simulink model "frb_stable_test"  (R2013b)
(part 3 of 48)

      mask help: This simple vector accumulator is based on a shift register. It outputs its previous accumulated vector after a new_acc pulse is received.
      mask init:
      | simple_bram_vacc_init(gcb, ...
      |     'vec_len', vec_len, ...
      |     'arith_type', arith_type, ...
      |     'n_bits', n_bits, ...
      |     'bin_pt', bin_pt);
      mask TypeOptions arith_type: Signed | Unsigned
  simple_bram_vacc45 : Subsystem  AncestorBlock=casper_library_accumulators/simple_bram_vacc  mask(simple_bram_vacc){vec_len=512, arith_type=Unsigned, n_bits=32, bin_pt=19}
      mask prompts: vec_len "Vector length:"; arith_type "Output type:"; n_bits "Bit width (output):"; bin_pt "Binary point (output):"
      mask help: This simple vector accumulator is based on a shift register. It outputs its previous accumulated vector after a new_acc pulse is received.
      mask init:
      | simple_bram_vacc_init(gcb, ...
      |     'vec_len', vec_len, ...
      |     'arith_type', arith_type, ...
      |     'n_bits', n_bits, ...
      |     'bin_pt', bin_pt);
      mask TypeOptions arith_type: Signed | Unsigned
  simple_bram_vacc46 : Subsystem  AncestorBlock=casper_library_accumulators/simple_bram_vacc  mask(simple_bram_vacc){vec_len=512, arith_type=Unsigned, n_bits=32, bin_pt=19}
      mask prompts: vec_len "Vector length:"; arith_type "Output type:"; n_bits "Bit width (output):"; bin_pt "Binary point (output):"
      mask help: This simple vector accumulator is based on a shift register. It outputs its previous accumulated vector after a new_acc pulse is received.
      mask init:
      | simple_bram_vacc_init(gcb, ...
      |     'vec_len', vec_len, ...
      |     'arith_type', arith_type, ...
      |     'n_bits', n_bits, ...
      |     'bin_pt', bin_pt);
      mask TypeOptions arith_type: Signed | Unsigned
  simple_bram_vacc5 : Subsystem  AncestorBlock=casper_library_accumulators/simple_bram_vacc  mask(simple_bram_vacc){vec_len=512, arith_type=Unsigned, n_bits=32, bin_pt=19}
      mask prompts: vec_len "Vector length:"; arith_type "Output type:"; n_bits "Bit width (output):"; bin_pt "Binary point (output):"
      mask help: This simple vector accumulator is based on a shift register. It outputs its previous accumulated vector after a new_acc pulse is received.
      mask init:
      | simple_bram_vacc_init(gcb, ...
      |     'vec_len', vec_len, ...
      |     'arith_type', arith_type, ...
      |     'n_bits', n_bits, ...
      |     'bin_pt', bin_pt);
      mask TypeOptions arith_type: Signed | Unsigned
  simple_bram_vacc6 : Subsystem  AncestorBlock=casper_library_accumulators/simple_bram_vacc  mask(simple_bram_vacc){vec_len=512, arith_type=Unsigned, n_bits=32, bin_pt=19}
      mask prompts: vec_len "Vector length:"; arith_type "Output type:"; n_bits "Bit width (output):"; bin_pt "Binary point (output):"
      mask help: This simple vector accumulator is based on a shift register. It outputs its previous accumulated vector after a new_acc pulse is received.
      mask init:
      | simple_bram_vacc_init(gcb, ...
      |     'vec_len', vec_len, ...
      |     'arith_type', arith_type, ...
      |     'n_bits', n_bits, ...
      |     'bin_pt', bin_pt);
      mask TypeOptions arith_type: Signed | Unsigned
  simple_bram_vacc7 : Subsystem  AncestorBlock=casper_library_accumulators/simple_bram_vacc  mask(simple_bram_vacc){vec_len=512, arith_type=Unsigned, n_bits=32, bin_pt=19}
      mask prompts: vec_len "Vector length:"; arith_type "Output type:"; n_bits "Bit width (output):"; bin_pt "Binary point (output):"
      mask help: This simple vector accumulator is based on a shift register. It outputs its previous accumulated vector after a new_acc pulse is received.
      mask init:
      | simple_bram_vacc_init(gcb, ...
      |     'vec_len', vec_len, ...
      |     'arith_type', arith_type, ...
      |     'n_bits', n_bits, ...
      |     'bin_pt', bin_pt);
      mask TypeOptions arith_type: Signed | Unsigned
  simple_bram_vacc8 : Subsystem  AncestorBlock=casper_library_accumulators/simple_bram_vacc  mask(simple_bram_vacc){vec_len=512, arith_type=Unsigned, n_bits=32, bin_pt=19}
      mask prompts: vec_len "Vector length:"; arith_type "Output type:"; n_bits "Bit width (output):"; bin_pt "Binary point (output):"
      mask help: This simple vector accumulator is based on a shift register. It outputs its previous accumulated vector after a new_acc pulse is received.
      mask init:
      | simple_bram_vacc_init(gcb, ...
      |     'vec_len', vec_len, ...
      |     'arith_type', arith_type, ...
      |     'n_bits', n_bits, ...
      |     'bin_pt', bin_pt);
      mask TypeOptions arith_type: Signed | Unsigned
  simple_bram_vacc9 : Subsystem  AncestorBlock=casper_library_accumulators/simple_bram_vacc  mask(simple_bram_vacc){vec_len=512, arith_type=Unsigned, n_bits=32, bin_pt=19}
      mask prompts: vec_len "Vector length:"; arith_type "Output type:"; n_bits "Bit width (output):"; bin_pt "Binary point (output):"
      mask help: This simple vector accumulator is based on a shift register. It outputs its previous accumulated vector after a new_acc pulse is received.
      mask init:
      | simple_bram_vacc_init(gcb, ...
      |     'vec_len', vec_len, ...
      |     'arith_type', arith_type, ...
      |     'n_bits', n_bits, ...
      |     'bin_pt', bin_pt);
      mask TypeOptions arith_type: Signed | Unsigned
  simple_bram_vacc_0a_1 : Subsystem  AncestorBlock=casper_library_accumulators/simple_bram_vacc  mask(simple_bram_vacc){vec_len=512, arith_type=Unsigned, n_bits=32, bin_pt=16}
      mask prompts: vec_len "Vector length:"; arith_type "Output type:"; n_bits "Bit width (output):"; bin_pt "Binary point (output):"
      mask help: This simple vector accumulator is based on a shift register. It outputs its previous accumulated vector after a new_acc pulse is received.
      mask init:
      | simple_bram_vacc_init(gcb, ...
      |     'vec_len', vec_len, ...
      |     'arith_type', arith_type, ...
      |     'n_bits', n_bits, ...
      |     'bin_pt', bin_pt);
      mask TypeOptions arith_type: Signed | Unsigned
  simple_bram_vacc_0a_2 : Subsystem  AncestorBlock=casper_library_accumulators/simple_bram_vacc  mask(simple_bram_vacc){vec_len=512, arith_type=Unsigned, n_bits=32, bin_pt=16}
      mask prompts: vec_len "Vector length:"; arith_type "Output type:"; n_bits "Bit width (output):"; bin_pt "Binary point (output):"
      mask help: This simple vector accumulator is based on a shift register. It outputs its previous accumulated vector after a new_acc pulse is received.
      mask init:
      | simple_bram_vacc_init(gcb, ...
      |     'vec_len', vec_len, ...
      |     'arith_type', arith_type, ...
      |     'n_bits', n_bits, ...
      |     'bin_pt', bin_pt);
      mask TypeOptions arith_type: Signed | Unsigned
  simple_bram_vacc_0a_3 : Subsystem  AncestorBlock=casper_library_accumulators/simple_bram_vacc  mask(simple_bram_vacc){vec_len=512, arith_type=Unsigned, n_bits=32, bin_pt=16}
      mask prompts: vec_len "Vector length:"; arith_type "Output type:"; n_bits "Bit width (output):"; bin_pt "Binary point (output):"
      mask help: This simple vector accumulator is based on a shift register. It outputs its previous accumulated vector after a new_acc pulse is received.
      mask init:
      | simple_bram_vacc_init(gcb, ...
      |     'vec_len', vec_len, ...
      |     'arith_type', arith_type, ...
      |     'n_bits', n_bits, ...
      |     'bin_pt', bin_pt);
      mask TypeOptions arith_type: Signed | Unsigned
  simple_bram_vacc_0a_8 : Subsystem  AncestorBlock=casper_library_accumulators/simple_bram_vacc  mask(simple_bram_vacc){vec_len=512, arith_type=Unsigned, n_bits=32, bin_pt=16}
      mask prompts: vec_len "Vector length:"; arith_type "Output type:"; n_bits "Bit width (output):"; bin_pt "Binary point (output):"
      mask help: This simple vector accumulator is based on a shift register. It outputs its previous accumulated vector after a new_acc pulse is received.
      mask init:
      | simple_bram_vacc_init(gcb, ...
      |     'vec_len', vec_len, ...
      |     'arith_type', arith_type, ...
      |     'n_bits', n_bits, ...
      |     'bin_pt', bin_pt);
      mask TypeOptions arith_type: Signed | Unsigned
  simple_bram_vacc_0c_16 : Subsystem  AncestorBlock=casper_library_accumulators/simple_bram_vacc  mask(simple_bram_vacc){vec_len=512, arith_type=Signed, n_bits=32, bin_pt=16}
      mask prompts: vec_len "Vector length:"; arith_type "Output type:"; n_bits "Bit width (output):"; bin_pt "Binary point (output):"
      mask help: This simple vector accumulator is based on a shift register. It outputs its previous accumulated vector after a new_acc pulse is received.
      mask init:
      | simple_bram_vacc_init(gcb, ...
      |     'vec_len', vec_len, ...
      |     'arith_type', arith_type, ...
      |     'n_bits', n_bits, ...
      |     'bin_pt', bin_pt);
      mask TypeOptions arith_type: Signed | Unsigned
  simple_bram_vacc_0c_17 : Subsystem  AncestorBlock=casper_library_accumulators/simple_bram_vacc  mask(simple_bram_vacc){vec_len=512, arith_type=Signed, n_bits=32, bin_pt=16}
      mask prompts: vec_len "Vector length:"; arith_type "Output type:"; n_bits "Bit width (output):"; bin_pt "Binary point (output):"
      mask help: This simple vector accumulator is based on a shift register. It outputs its previous accumulated vector after a new_acc pulse is received.
      mask init:
      | simple_bram_vacc_init(gcb, ...
      |     'vec_len', vec_len, ...
      |     'arith_type', arith_type, ...
      |     'n_bits', n_bits, ...
      |     'bin_pt', bin_pt);
      mask TypeOptions arith_type: Signed | Unsigned
  simple_bram_vacc_0c_18 : Subsystem  AncestorBlock=casper_library_accumulators/simple_bram_vacc  mask(simple_bram_vacc){vec_len=512, arith_type=Signed, n_bits=32, bin_pt=16}
      mask prompts: vec_len "Vector length:"; arith_type "Output type:"; n_bits "Bit width (output):"; bin_pt "Binary point (output):"
      mask help: This simple vector accumulator is based on a shift register. It outputs its previous accumulated vector after a new_acc pulse is received.
      mask init:
      | simple_bram_vacc_init(gcb, ...
      |     'vec_len', vec_len, ...
      |     'arith_type', arith_type, ...
      |     'n_bits', n_bits, ...
      |     'bin_pt', bin_pt);
      mask TypeOptions arith_type: Signed | Unsigned
  simple_bram_vacc_0c_19 : Subsystem  AncestorBlock=casper_library_accumulators/simple_bram_vacc  mask(simple_bram_vacc){vec_len=512, arith_type=Signed, n_bits=32, bin_pt=16}
      mask prompts: vec_len "Vector length:"; arith_type "Output type:"; n_bits "Bit width (output):"; bin_pt "Binary point (output):"
      mask help: This simple vector accumulator is based on a shift register. It outputs its previous accumulated vector after a new_acc pulse is received.
      mask init:
      | simple_bram_vacc_init(gcb, ...
      |     'vec_len', vec_len, ...
      |     'arith_type', arith_type, ...
      |     'n_bits', n_bits, ...
      |     'bin_pt', bin_pt);
      mask TypeOptions arith_type: Signed | Unsigned
  simple_bram_vacc_0c_20 : Subsystem  AncestorBlock=casper_library_accumulators/simple_bram_vacc  mask(simple_bram_vacc){vec_len=512, arith_type=Unsigned, n_bits=32, bin_pt=16}
      mask prompts: vec_len "Vector length:"; arith_type "Output type:"; n_bits "Bit width (output):"; bin_pt "Binary point (output):"
      mask help: This simple vector accumulator is based on a shift register. It outputs its previous accumulated vector after a new_acc pulse is received.
      mask init:
      | simple_bram_vacc_init(gcb, ...
      |     'vec_len', vec_len, ...
      |     'arith_type', arith_type, ...
      |     'n_bits', n_bits, ...
      |     'bin_pt', bin_pt);
      mask TypeOptions arith_type: Signed | Unsigned
  simple_bram_vacc_0c_21 : Subsystem  AncestorBlock=casper_library_accumulators/simple_bram_vacc  mask(simple_bram_vacc){vec_len=512, arith_type=Unsigned, n_bits=32, bin_pt=16}
      mask prompts: vec_len "Vector length:"; arith_type "Output type:"; n_bits "Bit width (output):"; bin_pt "Binary point (output):"
      mask help: This simple vector accumulator is based on a shift register. It outputs its previous accumulated vector after a new_acc pulse is received.
      mask init:
      | simple_bram_vacc_init(gcb, ...
      |     'vec_len', vec_len, ...
      |     'arith_type', arith_type, ...
      |     'n_bits', n_bits, ...
      |     'bin_pt', bin_pt);
      mask TypeOptions arith_type: Signed | Unsigned
  simple_bram_vacc_0c_22 : Subsystem  AncestorBlock=casper_library_accumulators/simple_bram_vacc  mask(simple_bram_vacc){vec_len=512, arith_type=Signed, n_bits=32, bin_pt=16}
      mask prompts: vec_len "Vector length:"; arith_type "Output type:"; n_bits "Bit width (output):"; bin_pt "Binary point (output):"
      mask help: This simple vector accumulator is based on a shift register. It outputs its previous accumulated vector after a new_acc pulse is received.
      mask init:
      | simple_bram_vacc_init(gcb, ...
      |     'vec_len', vec_len, ...
      |     'arith_type', arith_type, ...
      |     'n_bits', n_bits, ...
      |     'bin_pt', bin_pt);
      mask TypeOptions arith_type: Signed | Unsigned
  simple_bram_vacc_0c_23 : Subsystem  AncestorBlock=casper_library_accumulators/simple_bram_vacc  mask(simple_bram_vacc){vec_len=512, arith_type=Signed, n_bits=32, bin_pt=16}
      mask prompts: vec_len "Vector length:"; arith_type "Output type:"; n_bits "Bit width (output):"; bin_pt "Binary point (output):"
      mask help: This simple vector accumulator is based on a shift register. It outputs its previous accumulated vector after a new_acc pulse is received.
      mask init:
      | simple_bram_vacc_init(gcb, ...
      |     'vec_len', vec_len, ...
      |     'arith_type', arith_type, ...
      |     'n_bits', n_bits, ...
      |     'bin_pt', bin_pt);
      mask TypeOptions arith_type: Signed | Unsigned
  simple_bram_vacc_0c_4 : Subsystem  AncestorBlock=casper_library_accumulators/simple_bram_vacc  mask(simple_bram_vacc){vec_len=512, arith_type=Unsigned, n_bits=32, bin_pt=16}
      mask prompts: vec_len "Vector length:"; arith_type "Output type:"; n_bits "Bit width (output):"; bin_pt "Binary point (output):"
      mask help: This simple vector accumulator is based on a shift register. It outputs its previous accumulated vector after a new_acc pulse is received.
      mask init:
      | simple_bram_vacc_init(gcb, ...
      |     'vec_len', vec_len, ...
      |     'arith_type', arith_type, ...
      |     'n_bits', n_bits, ...
      |     'bin_pt', bin_pt);
      mask TypeOptions arith_type: Signed | Unsigned
  simple_bram_vacc_0c_5 : Subsystem  AncestorBlock=casper_library_accumulators/simple_bram_vacc  mask(simple_bram_vacc){vec_len=512, arith_type=Unsigned, n_bits=32, bin_pt=16}
      mask prompts: vec_len "Vector length:"; arith_type "Output type:"; n_bits "Bit width (output):"; bin_pt "Binary point (output):"
      mask help: This simple vector accumulator is based on a shift register. It outputs its previous accumulated vector after a new_acc pulse is received.
      mask init:
      | simple_bram_vacc_init(gcb, ...
      |     'vec_len', vec_len, ...
      |     'arith_type', arith_type, ...
      |     'n_bits', n_bits, ...
      |     'bin_pt', bin_pt);
      mask TypeOptions arith_type: Signed | Unsigned
  simple_bram_vacc_0c_6 : Subsystem  AncestorBlock=casper_library_accumulators/simple_bram_vacc  mask(simple_bram_vacc){vec_len=512, arith_type=Signed, n_bits=32, bin_pt=16}
      mask prompts: vec_len "Vector length:"; arith_type "Output type:"; n_bits "Bit width (output):"; bin_pt "Binary point (output):"
      mask help: This simple vector accumulator is based on a shift register. It outputs its previous accumulated vector after a new_acc pulse is received.
      mask init:
      | simple_bram_vacc_init(gcb, ...
      |     'vec_len', vec_len, ...
      |     'arith_type', arith_type, ...
      |     'n_bits', n_bits, ...
      |     'bin_pt', bin_pt);
      mask TypeOptions arith_type: Signed | Unsigned
  simple_bram_vacc_0c_7 : Subsystem  AncestorBlock=casper_library_accumulators/simple_bram_vacc  mask(simple_bram_vacc){vec_len=512, arith_type=Signed, n_bits=32, bin_pt=16}
      mask prompts: vec_len "Vector length:"; arith_type "Output type:"; n_bits "Bit width (output):"; bin_pt "Binary point (output):"
      mask help: This simple vector accumulator is based on a shift register. It outputs its previous accumulated vector after a new_acc pulse is received.
      mask init:
      | simple_bram_vacc_init(gcb, ...
      |     'vec_len', vec_len, ...
      |     'arith_type', arith_type, ...
      |     'n_bits', n_bits, ...
      |     'bin_pt', bin_pt);
      mask TypeOptions arith_type: Signed | Unsigned
  small_spec2 : Subsystem  Tag=xps:bram  AncestorBlock=xps_library/Shared_BRAM  mask{arith_type=Unsigned, addr_width=10, data_width=32, reg_prim_output=off, reg_core_output=off, optimization=Minimum_Area, data_bin_pt=0, init_vals=[0:2^10-1], sample_rate=1}
      mask prompts: arith_type "Output Data Type"; addr_width "Address width"; data_width "Data Width"; reg_prim_output "Register Primitive Output"; reg_core_output "Register Core Output"; data_bin_pt "Data Binary Point"; init_vals "Initial values (simulation only)"; sample_rate "Sample rate"
      mask init:
      | shared_bram_mask;
      mask TypeOptions arith_type: Unsigned | Signed  (2's comp)
      mask TypeOptions data_width: 8 | 16 | 32 | 64 | 128
      mask TypeOptions optimization: Minimum_Area | Low_Power
  snapshot : Subsystem  Tag=casper:snapshot  AncestorBlock=casper_library_scopes/snapshot  mask(snapshot){storage=bram, dram_dimm=1, dram_clock=200, nsamples=10, data_width=64, offset=off, circap=off, value=off, use_dsp48=off}
      mask prompts: storage "Storage medium"; dram_dimm "DRAM dimm"; dram_clock "DRAM clock rate"; nsamples "Number of Samples (2^?)"; data_width "Data width"; offset "Start delay support"; circap "Circular capture support"; value "Extra value capture support"; use_dsp48 "Use DSP48s to implement counters"
      mask help:
      | Standard snap block, but with the following optional extras;
      |  1) Optionally delay the fabric trigger by a user-specified number of valids.
      |  2) Capture continuously after a trigger until a stop pulse is received. Data is captured into BRAM continuously, with old data being overwritten until a stop command is received. Then stop capturing when memory is filled. This enables you to get some data before and some data after the stop pulse. Use the 'tr_en_cnt' register to determine where you are in your vector. 'Addr' register's MSb now indicates 'busy capturing'.
      |  3) Optionally capture a value on an input port to a register at the same time as the first data sample.
      |  4) Implement counters using DSP48Es to save resources.
      mask init: same as frb_stable_test/adcsnap1
      mask TypeOptions storage: bram | dram
      mask Callback storage: snapshot_callback();
      mask TypeOptions dram_dimm: 1 | 2 | 3 | 4
      mask TypeOptions dram_clock: 200 | 250 | 266 | 300 | 333
      mask TypeOptions data_width: 8 | 16 | 32 | 64 | 128
  spec1_0 : Subsystem  Tag=xps:bram  AncestorBlock=xps_library/Shared_BRAM  mask{arith_type=Unsigned, addr_width=9, data_width=64, reg_prim_output=on, reg_core_output=on, optimization=Minimum_Area, data_bin_pt=0, init_vals=[0:2^10-1], sample_rate=1}
      mask prompts: arith_type "Output Data Type"; addr_width "Address width"; data_width "Data Width"; reg_prim_output "Register Primitive Output"; reg_core_output "Register Core Output"; data_bin_pt "Data Binary Point"; init_vals "Initial values (simulation only)"; sample_rate "Sample rate"
      mask init:
      | shared_bram_mask;
      mask TypeOptions arith_type: Unsigned | Signed  (2's comp)
      mask TypeOptions data_width: 8 | 16 | 32 | 64 | 128
      mask TypeOptions optimization: Minimum_Area | Low_Power
  spec1_1 : Subsystem  Tag=xps:bram  AncestorBlock=xps_library/Shared_BRAM  mask{arith_type=Unsigned, addr_width=9, data_width=64, reg_prim_output=on, reg_core_output=on, optimization=Minimum_Area, data_bin_pt=0, init_vals=[0:2^10-1], sample_rate=1}
      mask prompts: arith_type "Output Data Type"; addr_width "Address width"; data_width "Data Width"; reg_prim_output "Register Primitive Output"; reg_core_output "Register Core Output"; data_bin_pt "Data Binary Point"; init_vals "Initial values (simulation only)"; sample_rate "Sample rate"
      mask init:
      | shared_bram_mask;
      mask TypeOptions arith_type: Unsigned | Signed  (2's comp)
      mask TypeOptions data_width: 8 | 16 | 32 | 64 | 128
      mask TypeOptions optimization: Minimum_Area | Low_Power
  spec2_0 : Subsystem  Tag=xps:bram  AncestorBlock=xps_library/Shared_BRAM  mask{arith_type=Unsigned, addr_width=9, data_width=64, reg_prim_output=on, reg_core_output=on, optimization=Minimum_Area, data_bin_pt=0, init_vals=[0:2^10-1], sample_rate=1}
      mask prompts: arith_type "Output Data Type"; addr_width "Address width"; data_width "Data Width"; reg_prim_output "Register Primitive Output"; reg_core_output "Register Core Output"; data_bin_pt "Data Binary Point"; init_vals "Initial values (simulation only)"; sample_rate "Sample rate"
      mask init:
      | shared_bram_mask;
      mask TypeOptions arith_type: Unsigned | Signed  (2's comp)
      mask TypeOptions data_width: 8 | 16 | 32 | 64 | 128
      mask TypeOptions optimization: Minimum_Area | Low_Power
  spec2_1 : Subsystem  Tag=xps:bram  AncestorBlock=xps_library/Shared_BRAM  mask{arith_type=Unsigned, addr_width=9, data_width=64, reg_prim_output=on, reg_core_output=on, optimization=Minimum_Area, data_bin_pt=0, init_vals=[0:2^10-1], sample_rate=1}
      mask prompts: arith_type "Output Data Type"; addr_width "Address width"; data_width "Data Width"; reg_prim_output "Register Primitive Output"; reg_core_output "Register Core Output"; data_bin_pt "Data Binary Point"; init_vals "Initial values (simulation only)"; sample_rate "Sample rate"
      mask init:
      | shared_bram_mask;
      mask TypeOptions arith_type: Unsigned | Signed  (2's comp)
      mask TypeOptions data_width: 8 | 16 | 32 | 64 | 128
      mask TypeOptions optimization: Minimum_Area | Low_Power
  spec3_0 : Subsystem  Tag=xps:bram  AncestorBlock=xps_library/Shared_BRAM  mask{arith_type=Unsigned, addr_width=9, data_width=64, reg_prim_output=on, reg_core_output=on, optimization=Minimum_Area, data_bin_pt=0, init_vals=[0:2^10-1], sample_rate=1}
      mask prompts: arith_type "Output Data Type"; addr_width "Address width"; data_width "Data Width"; reg_prim_output "Register Primitive Output"; reg_core_output "Register Core Output"; data_bin_pt "Data Binary Point"; init_vals "Initial values (simulation only)"; sample_rate "Sample rate"
      mask init:
      | shared_bram_mask;
      mask TypeOptions arith_type: Unsigned | Signed  (2's comp)
      mask TypeOptions data_width: 8 | 16 | 32 | 64 | 128
      mask TypeOptions optimization: Minimum_Area | Low_Power
  spec3_1 : Subsystem  Tag=xps:bram  AncestorBlock=xps_library/Shared_BRAM  mask{arith_type=Unsigned, addr_width=9, data_width=64, reg_prim_output=on, reg_core_output=on, optimization=Minimum_Area, data_bin_pt=0, init_vals=[0:2^10-1], sample_rate=1}
      mask prompts: arith_type "Output Data Type"; addr_width "Address width"; data_width "Data Width"; reg_prim_output "Register Primitive Output"; reg_core_output "Register Core Output"; data_bin_pt "Data Binary Point"; init_vals "Initial values (simulation only)"; sample_rate "Sample rate"
      mask init:
      | shared_bram_mask;
      mask TypeOptions arith_type: Unsigned | Signed  (2's comp)
      mask TypeOptions data_width: 8 | 16 | 32 | 64 | 128
      mask TypeOptions optimization: Minimum_Area | Low_Power
  spec4_0 : Subsystem  Tag=xps:bram  AncestorBlock=xps_library/Shared_BRAM  mask{arith_type=Unsigned, addr_width=9, data_width=64, reg_prim_output=on, reg_core_output=on, optimization=Minimum_Area, data_bin_pt=0, init_vals=[0:2^10-1], sample_rate=1}
      mask prompts: arith_type "Output Data Type"; addr_width "Address width"; data_width "Data Width"; reg_prim_output "Register Primitive Output"; reg_core_output "Register Core Output"; data_bin_pt "Data Binary Point"; init_vals "Initial values (simulation only)"; sample_rate "Sample rate"
      mask init:
      | shared_bram_mask;
      mask TypeOptions arith_type: Unsigned | Signed  (2's comp)
      mask TypeOptions data_width: 8 | 16 | 32 | 64 | 128
      mask TypeOptions optimization: Minimum_Area | Low_Power
  spec4_1 : Subsystem  Tag=xps:bram  AncestorBlock=xps_library/Shared_BRAM  mask{arith_type=Unsigned, addr_width=9, data_width=64, reg_prim_output=on, reg_core_output=on, optimization=Minimum_Area, data_bin_pt=0, init_vals=[0:2^10-1], sample_rate=1}
      mask prompts: arith_type "Output Data Type"; addr_width "Address width"; data_width "Data Width"; reg_prim_output "Register Primitive Output"; reg_core_output "Register Core Output"; data_bin_pt "Data Binary Point"; init_vals "Initial values (simulation only)"; sample_rate "Sample rate"
      mask init:
      | shared_bram_mask;
      mask TypeOptions arith_type: Unsigned | Signed  (2's comp)
      mask TypeOptions data_width: 8 | 16 | 32 | 64 | 128
      mask TypeOptions optimization: Minimum_Area | Low_Power
  sync_gen : Subsystem  AncestorBlock=casper_library_misc/sync_gen  mask(sync_gen){sim_acc_len=1, fft_size=4096, fft_simult_inputs=8, pfb_fir_taps=3, reorder_vec=[2 2 9], scale=1}
      mask prompts: sim_acc_len "Simulation Accumulation Length"; fft_size "FFT Size"; fft_simult_inputs "Simultaneous Inputs (FFT)"; pfb_fir_taps "Taps in pfb_fir (use 1 if no pfb_fir)"; reorder_vec "Reorder Orders (e.g. [2 2 2])"
      mask help:
      | This block computes the sync period based on system parameters as
      | described in Casper memo.  Detailed descritions of the block's
      | variables can be found in the 'Block Documentation' section of
      | the CASPER wiki.
      mask init:
      | sync_gen_init(gcb, ...
      |     'sim_acc_len', sim_acc_len, ...
      |     'fft_size', fft_size, ...
      |     'fft_simult_inputs', fft_simult_inputs,...
      |     'pfb_fir_taps', pfb_fir_taps, ...
      |     'reorder_vec', reorder_vec, ...
      |     'scale', scale);
      settings: AttributesFormatString=sim_sync_period=27648
      mask Help:
      | SyncPeriod=LCM(reorder_vec)*(acc_num)*(pfb_fir_len)*(fft_size/fft_simult_inputs)
      | 
      | See CASPER sync pulse memo for more details.
  sync_tree2 : Subsystem
  ten_Gbe_v2 : Subsystem  Tag=xps:tengbe_v2  AncestorBlock=xps_library/ten_Gbe_v2  mask(ten_GbE_v2){flavour=sfp+, slot=0, port_r1=0, port_r2_cx4=0, port_r2_sfpp=0, rx_dist_ram=off, large_frames=on, show_param=on, pre_emph_r2=1.07, pre_emph=3, post_emph_r2=0.18, rxeqmix_r2=7, swing_r2=940, swing=800, fab_en=on, fab_mac=hex2dec('123456780000'), fab_ip=192*(2^24) + 168*(2^16) + 5*(2^8) + 20*(2^0), fab_udp=10000, fab_gate=1, cpu_rx_en=off, cpu_tx_en=on, ttl=hex2dec('FF'), promisc_mode=off, debug_ctr_width=16, txctr=on, txerrctr=on, txerrctr_len=100, txofctr=on, txfullctr=on, txvldctr=on, txsnaplen=16384, rxctr=off, rxerrctr=off, rxerrctr_len=100, rxofctr=off, rxbadctr=off, rxvldctr=off, rxeofctr=off, rxsnaplen=0 - no snap}
      mask prompts: flavour "Mezzanine card flavour"; slot "Card slot"; port_r1 "Port"; port_r2_cx4 "Port"; port_r2_sfpp "Port"; rx_dist_ram "Shallow RX Fifo (Beware overruns!)"; large_frames "Enable Large TX Frames (8k+512)"; show_param "---------------------- Show Implementation Parameters -----------------------------------------------------------------------------------"; pre_emph_r2 "Pre-emphasis (dB)"; pre_emph "Pre-emphasis"; post_emph_r2 "Post-emphasis (dB)"; rxeqmix_r2 "Receive equalisation"; swing_r2 "Driver Swing Control (mVppd)"; swing "Differential swing"; fab_en "Enable fabric on startup"; fab_mac "Fabric MAC Address"; fab_ip "Fabric IP Address"; fab_udp "Fabric UDP Port"; fab_gate "Fabric Gateway"; cpu_rx_en "Enable CPU RX"; cpu_tx_en "Enable CPU TX"; promisc_mode "Promiscuous mode"; debug_ctr_width "Debug counter width"; txctr "TX - core_txctr"; txerrctr "TX packet length error - core_txerrctr"; txerrctr_len "-- expected TX packet length"; txofctr "TX overflow - core_txofctr"; txfullctr "TX full - core_txfullctr"; txvldctr "TX valid cycle - core_txvldctr"; txsnaplen "TX snapshot length"; rxctr "RX - core_rxctr"; rxerrctr "RX packet length error - core_rxerrctr"; rxerrctr_len "-- expected RX packet length"; rxofctr "RX overflow - core_rxofctr"; rxbadctr "RX bad - core_rxbadctr"; rxvldctr "RX valid cycle - core_rxvldctr"; rxeofctr "RX eof - core_rxeofctr"; rxsnaplen "RX snapshot length"
      mask help: This block sends and receives UDP frames (packets). It accepts a 64 bit wide data stream with user-determined frame breaks. The data stream is wrapped in a UDP frame for transmission. Incoming UDP packets are unwrapped and the data presented as a 64 bit wide stream.
      mask init:
      | temp = eval(get_param(gcb, 'debug_ctr_width'));
      | if temp <= 0,
      |     error('Debug counters cannot be ltoet zero.');
      | end
      | tengbe_v2_mask(gcb)
      mask TypeOptions flavour: sfp+ | cx4
      mask Callback flavour: tengbe_v2_callback
      mask TypeOptions slot: 0 | 1
      mask TypeOptions port_r1: 0 | 1 | 2 | 3
      mask TypeOptions port_r2_cx4: 0 | 1 | 2
      mask TypeOptions port_r2_sfpp: 0 | 1 | 2 | 3
      mask Callback show_param: tengbe_v2_callback
      mask TypeOptions pre_emph_r2: 0.15 | 0.3 | 0.45 | 0.61 | 0.74 | 0.91 | 1.07 | 1.25 | 1.36 | 1.55 | 1.74 | 1.94 | 2.11 | 2.32 | 2.54 | 2.77
      mask TypeOptions pre_emph: 0 | 1 | 2 | 3
      mask TypeOptions post_emph_r2: 0.18 | 0.19 | 0.2 | 0.39 | 0.63 | 0.82 | 1.07 | 1.32 | 1.6 | 1.65 | 1.94 | 2.21 | 2.52 | 2.76 | 3.08 | 3.41 | 3.77 | 3.97 | 4.36 | 4.73 | 5.16 | 5.47 | 5.93 | 6.38 | 6.89
      mask TypeOptions rxeqmix_r2: 0 | 1 | 2 | 3 | 4 | 5 | 6 | 7
      mask TypeOptions swing_r2: 110 | 210 | 310 | 400 | 480 | 570 | 660 | 740 | 810 | 880 | 940 | 990 | 1040 | 1080 | 1110 | 1130
      mask TypeOptions swing: 400 | 500 | 600 | 700 | 800
      mask Callback txerrctr:
      | blk = gcb;
      | mask_visibilities = get_param(blk, 'MaskVisibilities');
      | mask_names = get_param(blk, 'MaskNames');
      | if strcmp(get_param(blk, 'txerrctr'), 'on')
      |     mask_visibilities{ismember(mask_names, 'txerrctr_len')} = 'on';
      | else
      |     mask_visibilities{ismember(mask_names, 'txerrctr_len')} = 'off';
      | end
      | set_param(blk, 'MaskVisibilities', mask_visibilities);
      mask TypeOptions txsnaplen: 0 - no snap | 256 | 512 | 1024 | 2048 | 4096 | 8192 | 16384
      mask Callback rxerrctr:
      | blk = gcb;
      | mask_visibilities = get_param(blk, 'MaskVisibilities');
      | mask_names = get_param(blk, 'MaskNames');
      | if strcmp(get_param(blk, 'rxerrctr'), 'on')
      |     mask_visibilities{ismember(mask_names, 'rxerrctr_len')} = 'on';
      | else
      |     mask_visibilities{ismember(mask_names, 'rxerrctr_len')} = 'off';
      | end
      | set_param(blk, 'MaskVisibilities', mask_visibilities);
      mask TypeOptions rxsnaplen: 0 - no snap | 256 | 512 | 1024 | 2048 | 4096 | 8192 | 16384
  theta : Subsystem  Tag=xps:sw_reg  AncestorBlock=xps_library/software_register  mask(swreg){io_dir=From Processor, io_delay=0, sample_period=1, names=reg, bitwidths=32, bin_pts=0, arith_types=0, sim_port=on, show_format=on}
      mask prompts: io_dir "I/O direction"; io_delay "I/O delay"; sample_period "Sample period"; names "Bitfield names [msb...lsb]"; bitwidths "Bitfield widths"; bin_pts "Bitfield binary pts"; arith_types "Bitfield types, ufix=0, fix=1, bool=2"; sim_port "Provide sim input/output?"; show_format "Print format string?"
      mask help: A 32-bit software-accessible register. Can be divided into bitfields of varying widths and types using the fields in the block mask.
      mask init:
      | try
      |     swreg_init(gcb)
      | catch ex
      |     disp(sprintf('%s: %s', gcb, ex.message))
      |     errordlg(ex.message)
      | end
      settings: AttributesFormatString=1input:uf32.0 = 32 bits
      mask TypeOptions io_dir: To Processor | From Processor
      mask Callback io_dir:
      | mask_enables = get_param(gcb, 'MaskEnables');
      | mask_names = get_param(gcb, 'MaskNames');
      | if strcmp(get_param(gcb, 'io_dir'), 'To Processor'),
      |     mask_enables{ismember(mask_names, 'sample_period')} = 'off';
      | else
      |     mask_enables{ismember(mask_names, 'sample_period')} = 'on';
      | end
      | set_param(gcb, 'MaskEnables', mask_enables);
  thresh0 : Subsystem  Tag=xps:bram  AncestorBlock=xps_library/Shared_BRAM  mask{arith_type=Unsigned, addr_width=10, data_width=32, reg_prim_output=off, reg_core_output=off, optimization=Minimum_Area, data_bin_pt=0, init_vals=[0:2^10-1], sample_rate=1}
      mask prompts: arith_type "Output Data Type"; addr_width "Address width"; data_width "Data Width"; reg_prim_output "Register Primitive Output"; reg_core_output "Register Core Output"; data_bin_pt "Data Binary Point"; init_vals "Initial values (simulation only)"; sample_rate "Sample rate"
      mask init:
      | shared_bram_mask;
      mask TypeOptions arith_type: Unsigned | Signed  (2's comp)
      mask TypeOptions data_width: 8 | 16 | 32 | 64 | 128
      mask TypeOptions optimization: Minimum_Area | Low_Power
  thresh1 : Subsystem  Tag=xps:bram  AncestorBlock=xps_library/Shared_BRAM  mask{arith_type=Unsigned, addr_width=10, data_width=32, reg_prim_output=off, reg_core_output=off, optimization=Minimum_Area, data_bin_pt=0, init_vals=[0:2^10-1], sample_rate=1}
      mask prompts: arith_type "Output Data Type"; addr_width "Address width"; data_width "Data Width"; reg_prim_output "Register Primitive Output"; reg_core_output "Register Core Output"; data_bin_pt "Data Binary Point"; init_vals "Initial values (simulation only)"; sample_rate "Sample rate"
      mask init:
      | shared_bram_mask;
      mask TypeOptions arith_type: Unsigned | Signed  (2's comp)
      mask TypeOptions data_width: 8 | 16 | 32 | 64 | 128
      mask TypeOptions optimization: Minimum_Area | Low_Power
  thresh2 : Subsystem  Tag=xps:bram  AncestorBlock=xps_library/Shared_BRAM  mask{arith_type=Unsigned, addr_width=10, data_width=32, reg_prim_output=off, reg_core_output=off, optimization=Minimum_Area, data_bin_pt=0, init_vals=[0:2^10-1], sample_rate=1}
      mask prompts: arith_type "Output Data Type"; addr_width "Address width"; data_width "Data Width"; reg_prim_output "Register Primitive Output"; reg_core_output "Register Core Output"; data_bin_pt "Data Binary Point"; init_vals "Initial values (simulation only)"; sample_rate "Sample rate"
      mask init:
      | shared_bram_mask;
      mask TypeOptions arith_type: Unsigned | Signed  (2's comp)
      mask TypeOptions data_width: 8 | 16 | 32 | 64 | 128
      mask TypeOptions optimization: Minimum_Area | Low_Power
  thresh3 : Subsystem  Tag=xps:bram  AncestorBlock=xps_library/Shared_BRAM  mask{arith_type=Unsigned, addr_width=10, data_width=32, reg_prim_output=off, reg_core_output=off, optimization=Minimum_Area, data_bin_pt=0, init_vals=[0:2^10-1], sample_rate=1}
      mask prompts: arith_type "Output Data Type"; addr_width "Address width"; data_width "Data Width"; reg_prim_output "Register Primitive Output"; reg_core_output "Register Core Output"; data_bin_pt "Data Binary Point"; init_vals "Initial values (simulation only)"; sample_rate "Sample rate"
      mask init:
      | shared_bram_mask;
      mask TypeOptions arith_type: Unsigned | Signed  (2's comp)
      mask TypeOptions data_width: 8 | 16 | 32 | 64 | 128
      mask TypeOptions optimization: Minimum_Area | Low_Power
  thresh_offset : Subsystem  Tag=xps:sw_reg  AncestorBlock=xps_library/software_register  mask(swreg){io_dir=From Processor, io_delay=0, sample_period=1, names=reg, bitwidths=32, bin_pts=0, arith_types=0, sim_port=on, show_format=on}
      mask prompts: io_dir "I/O direction"; io_delay "I/O delay"; sample_period "Sample period"; names "Bitfield names [msb...lsb]"; bitwidths "Bitfield widths"; bin_pts "Bitfield binary pts"; arith_types "Bitfield types, ufix=0, fix=1, bool=2"; sim_port "Provide sim input/output?"; show_format "Print format string?"
      mask help: A 32-bit software-accessible register. Can be divided into bitfields of varying widths and types using the fields in the block mask.
      mask init:
      | try
      |     swreg_init(gcb)
      | catch ex
      |     disp(sprintf('%s: %s', gcb, ex.message))
      |     errordlg(ex.message)
      | end
      settings: AttributesFormatString=1input:uf32.0 = 32 bits
      mask TypeOptions io_dir: To Processor | From Processor
      mask Callback io_dir:
      | mask_enables = get_param(gcb, 'MaskEnables');
      | mask_names = get_param(gcb, 'MaskNames');
      | if strcmp(get_param(gcb, 'io_dir'), 'To Processor'),
      |     mask_enables{ismember(mask_names, 'sample_period')} = 'off';
      | else
      |     mask_enables{ismember(mask_names, 'sample_period')} = 'on';
      | end
      | set_param(gcb, 'MaskEnables', mask_enables);
  ucf : xps_library/ucf  Tag=xps:ucf  ucf_file=/home/seba/frb_stable/one_gbe_pblock.ucf
  var0 : Subsystem  Tag=xps:bram  AncestorBlock=xps_library/Shared_BRAM  mask{arith_type=Unsigned, addr_width=10, data_width=64, reg_prim_output=off, reg_core_output=off, optimization=Minimum_Area, data_bin_pt=0, init_vals=[0:2^10-1], sample_rate=1}
      mask prompts: arith_type "Output Data Type"; addr_width "Address width"; data_width "Data Width"; reg_prim_output "Register Primitive Output"; reg_core_output "Register Core Output"; data_bin_pt "Data Binary Point"; init_vals "Initial values (simulation only)"; sample_rate "Sample rate"
      mask init:
      | shared_bram_mask;
      mask TypeOptions arith_type: Unsigned | Signed  (2's comp)
      mask TypeOptions data_width: 8 | 16 | 32 | 64 | 128
      mask TypeOptions optimization: Minimum_Area | Low_Power
  wires:
  cnt_rst/1(in_reg) -> pipeline5/1(d)
  Slice/1 -> [cnt_rst]
  acc_len/1(in_reg) -> pipeline6/1(d)
  pipeline6/1(q) -> [acc_len]
  sync_gen/1(sync_out) -> pipeline143/1(d)
  pipeline143/1(q) -> [sync_gen]
  gain/1(in_reg) -> pipeline31/1(d)
  pipeline31/1(q) -> [gain]
  gain_adc/1(in_reg) -> pipeline14/1(d)
  pipeline14/1(q) -> [gain_adc]
  Slice3/1 -> pipeline54/1(d)
  pipeline54/1(q) -> [rst_detect]
  [sync_gen] -> pipeline41/1(d)
  asiaa_adc5g1/17(sync_out) -> Terminator6/1
  conv_bus1/1(q0) -> pipeline301/1
  conv_bus1/2(q1) -> pipeline349/1
  conv_bus1/3(q2) -> pipeline399/1
  conv_bus1/4(q3) -> pipeline400/1
  conv_bus1/5(q4) -> pipeline401/1
  conv_bus1/6(q5) -> pipeline402/1
  conv_bus1/7(q6) -> pipeline300/1
  conv_bus1/8(q7) -> pipeline299/1
  Black Box6/6 -> Terminator7/1
  Black Box6/1 -> Delay37/1
  Black Box6/2 -> Delay35/1
  Black Box6/3 -> Delay58/1
  Black Box6/4 -> Delay59/1
  Black Box6/5 -> Delay60/1
  bus_create1/1(bus_out) -> pipeline599/1(d)
  Constant123/1 -> adcsnap1/3(trig), adcsnap1/2(we)
  pipeline599/1(q) -> adcsnap1/1(din)
  Delay57/1 -> Delay68/1
  power7/1 -> Delay71/1
  power5/1 -> Delay69/1
  power4/1 -> Delay67/1
  power6/1 -> Delay70/1
  Delay71/1 -> Shift36/1
  Delay69/1 -> Shift34/1
  Delay66/1 -> acc_cntrl11/2(sync)
  [acc_len] -> pipeline22/1
  [cnt_rst] -> pipeline12/1
  Delay72/1 -> pipeline304/1(d)
  pipeline315/1(q) -> simple_bram_vacc46/1(new_acc)
  pipeline311/1(q) -> simple_bram_vacc46/2(din)
  pipeline314/1(q) -> pipeline105/1(d)
  acc_cntrl11/1(new_acc) -> pipeline398/1(d)
  pipeline304/1(q) -> pipeline394/1(d)
  simple_bram_vacc46/1(dout) -> pipeline97/1(d)
  spec1_0/1(data_out) -> Terminator46/1
  simple_bram_vacc46/2(valid) -> pipeline98/1(d)
  pipeline305/1(q) -> simple_bram_vacc43/1(new_acc)
  pipeline303/1(q) -> simple_bram_vacc43/2(din)
  simple_bram_vacc43/1(dout) -> pipeline99/1(d)
  spec1_1/1(data_out) -> Terminator43/1
  pipeline309/1(q) -> simple_bram_vacc45/1(new_acc)
  pipeline308/1(q) -> simple_bram_vacc45/2(din)
  simple_bram_vacc45/1(dout) -> pipeline101/1(d)
  pipeline307/1(q) -> simple_bram_vacc44/1(new_acc)
  pipeline306/1(q) -> simple_bram_vacc44/2(din)
  simple_bram_vacc44/1(dout) -> pipeline103/1(d)
  simple_bram_vacc44/2(valid) -> pipeline28/1(d)
  Delay73/1 -> pipeline310/1(d)
  pipeline310/1(q) -> pipeline395/1(d)
  Delay64/1 -> pipeline312/1(d)
  pipeline312/1(q) -> pipeline396/1(d)
  Delay65/1 -> pipeline313/1(d)
  pipeline313/1(q) -> pipeline397/1(d)
  Delay68/1 -> Delay48/1
  Delay67/1 -> Shift33/1
  Delay70/1 -> Shift35/1
  pipeline397/1(q) -> pipeline306/1(d)
  pipeline394/1(q) -> pipeline311/1(d)
  pipeline396/1(q) -> pipeline308/1(d)
  pipeline395/1(q) -> pipeline303/1(d)
  pipeline398/1(q) -> pipeline314/1(d), pipeline307/1(d), pipeline309/1(d), pipeline305/1(d), pipeline315/1(d)
  pipeline298/1 -> bus_expand/1(bus_in)
  conv_bus1/9(q8) -> pipeline298/1, [adc0_a_red]
  pipeline299/1 -> pipeline40/1(d), bus_create1/8(in8)
  pipeline300/1 -> pipeline39/1(d), bus_create1/7(in7)
  pipeline301/1 -> pipeline32/1(d), bus_create1/1(in1)
  pipeline349/1 -> pipeline33/1(d), bus_create1/2(in2)
  pipeline399/1 -> pipeline34/1(d), bus_create1/3(in3)
  pipeline400/1 -> pipeline36/1(d), bus_create1/4(in4)
  pipeline401/1 -> pipeline37/1(d), bus_create1/5(in5)
  pipeline402/1 -> pipeline38/1(d), bus_create1/6(in6)
  asiaa_adc5g1/6(a5) -> conv_bus1/7(i5)
  asiaa_adc5g1/4(a3) -> conv_bus1/5(i3)
  asiaa_adc5g1/1(a0) -> conv_bus1/2(i0)
  asiaa_adc5g1/5(a4) -> conv_bus1/6(i4)
  asiaa_adc5g1/2(a1) -> conv_bus1/3(i1)
  asiaa_adc5g1/3(a2) -> conv_bus1/4(i2)
  asiaa_adc5g1/7(a6) -> conv_bus1/8(i6)
  asiaa_adc5g1/8(a7) -> conv_bus1/9(i7)
  asiaa_adc5g1/10(c1) -> conv_bus2/3(i1)
  asiaa_adc5g1/11(c2) -> conv_bus2/4(i2)
  asiaa_adc5g1/12(c3) -> conv_bus2/5(i3)
  asiaa_adc5g1/13(c4) -> conv_bus2/6(i4)
  asiaa_adc5g1/14(c5) -> conv_bus2/7(i5)
  asiaa_adc5g1/15(c6) -> conv_bus2/8(i6)
  asiaa_adc5g1/16(c7) -> conv_bus2/9(i7)
  [gain_adc] -> pipeline272/1
  Constant6/1 -> snapshot/2(we), snapshot/3(trig)
  bus_expand/1(msb_out8) -> Convert4/1
  bus_expand/2(out7) -> Convert5/1
  bus_expand/3(out6) -> Convert6/1
  bus_expand/4(out5) -> Convert7/1
  bus_expand/5(out4) -> Convert8/1
  bus_expand/6(out3) -> Convert9/1
  bus_expand/7(out2) -> Convert10/1
  bus_expand/8(lsb_out1) -> Convert11/1
  Convert11/1 -> bus_create2/8(in8)
  Convert10/1 -> bus_create2/7(in7)
  Convert9/1 -> bus_create2/6(in6)
  Convert8/1 -> bus_create2/5(in5)
  Convert7/1 -> bus_create2/4(in4)
  Convert6/1 -> bus_create2/3(in3)
  Convert5/1 -> bus_create2/2(in2)
  Convert4/1 -> bus_create2/1(in1)
  bus_create2/1(bus_out) -> snapshot/1(din)
  [sync_gen] -> pipeline63/1(d)
  Delay86/1 -> Delay90/1, [fft1_sync]
  Delay85/1 -> [fft1_ch0], power1/1
  conv_bus2/1(q0) -> pipeline42/1
  conv_bus2/2(q1) -> pipeline47/1
  conv_bus2/3(q2) -> pipeline58/1
  conv_bus2/4(q3) -> pipeline60/1
  conv_bus2/5(q4) -> pipeline61/1
  conv_bus2/6(q5) -> pipeline62/1
  conv_bus2/7(q6) -> pipeline11/1
  conv_bus2/8(q7) -> pipeline10/1
  Delay94/1 -> [fft1_ch1], power2/1
  Delay95/1 -> [fft1_ch2], power3/1
  Delay96/1 -> [fft1_ch3], power8/1
  bus_create3/1(bus_out) -> pipeline64/1(d)
  Constant11/1 -> adcsnap2/3(trig), adcsnap2/2(we)
  pipeline64/1(q) -> adcsnap2/1(din)
  Delay90/1 -> Delay106/1
  power8/1 -> Delay110/1
  power2/1 -> Delay108/1
  power1/1 -> Delay107/1
  power3/1 -> Delay109/1
  conv_bus2/9(q8) -> [adc0_c_red]
  pipeline10/1 -> pipeline59/1(d), bus_create3/8(in8)
  pipeline11/1 -> pipeline57/1(d), bus_create3/7(in7)
  pipeline42/1 -> pipeline43/1(d), bus_create3/1(in1)
  pipeline47/1 -> pipeline44/1(d), bus_create3/2(in2)
  pipeline58/1 -> pipeline46/1(d), bus_create3/3(in3)
  pipeline60/1 -> pipeline48/1(d), bus_create3/4(in4)
  pipeline61/1 -> pipeline55/1(d), bus_create3/5(in5)
  pipeline62/1 -> pipeline56/1(d), bus_create3/6(in6)
  [gain_adc] -> pipeline273/1
  asiaa_adc5g1/9(c0) -> conv_bus2/2(i0)
  Delay103/1 -> acc_cntrl3/2(sync)
  [acc_len] -> pipeline26/1
  [cnt_rst] -> pipeline51/1
  Delay104/1 -> pipeline66/1(d)
  pipeline77/1(q) -> simple_bram_vacc7/1(new_acc)
  pipeline73/1(q) -> simple_bram_vacc7/2(din)
  pipeline76/1(q) -> pipeline88/1(d)
  acc_cntrl3/1(new_acc) -> pipeline82/1(d)
  pipeline66/1(q) -> pipeline78/1(d)
  simple_bram_vacc7/1(dout) -> pipeline89/1(d)
  simple_bram_vacc7/2(valid) -> pipeline90/1(d)
  pipeline67/1(q) -> simple_bram_vacc1/1(new_acc)
  pipeline65/1(q) -> simple_bram_vacc1/2(din)
  simple_bram_vacc1/1(dout) -> pipeline91/1(d)
  simple_bram_vacc1/2(valid) -> pipeline92/1(d)
  pipeline71/1(q) -> simple_bram_vacc6/1(new_acc)
  pipeline70/1(q) -> simple_bram_vacc6/2(din)
  simple_bram_vacc6/1(dout) -> pipeline93/1(d)
  pipeline69/1(q) -> simple_bram_vacc5/1(new_acc)
  pipeline68/1(q) -> simple_bram_vacc5/2(din)
  simple_bram_vacc5/1(dout) -> pipeline95/1(d)
  simple_bram_vacc5/2(valid) -> pipeline96/1(d)
  Delay105/1 -> pipeline72/1(d)
  pipeline72/1(q) -> pipeline79/1(d)
  Delay101/1 -> pipeline74/1(d)
  pipeline74/1(q) -> pipeline80/1(d)
  Delay102/1 -> pipeline75/1(d)
  pipeline75/1(q) -> pipeline81/1(d)
  pipeline81/1(q) -> pipeline68/1(d)
  pipeline78/1(q) -> pipeline73/1(d)
  pipeline80/1(q) -> pipeline70/1(d)
  pipeline79/1(q) -> pipeline65/1(d)
  pipeline82/1(q) -> pipeline76/1(d), pipeline69/1(d), pipeline71/1(d), pipeline67/1(d), pipeline77/1(d)
  pipeline88/1(q) -> Counter5/1
  pipeline89/1(q) -> Reinterpret4/1
  pipeline91/1(q) -> Reinterpret8/1
  pipeline93/1(q) -> Reinterpret9/1
  pipeline95/1(q) -> Reinterpret10/1
  pipeline97/1(q) -> Reinterpret40/1
  pipeline98/1(q) -> Counter22/2
  pipeline99/1(q) -> Reinterpret41/1
  pipeline101/1(q) -> Reinterpret42/1
  pipeline103/1(q) -> Reinterpret43/1
  pipeline105/1(q) -> Counter22/1
  asiaa_adc5g/17(sync_out) -> Terminator12/1
  asiaa_adc5g/6(a5) -> conv_bus3/7(i5)
  asiaa_adc5g/4(a3) -> conv_bus3/5(i3)
  asiaa_adc5g/1(a0) -> conv_bus3/2(i0)
  asiaa_adc5g/5(a4) -> conv_bus3/6(i4)
  asiaa_adc5g/2(a1) -> conv_bus3/3(i1)
  asiaa_adc5g/3(a2) -> conv_bus3/4(i2)
  asiaa_adc5g/7(a6) -> conv_bus3/8(i6)
  asiaa_adc5g/8(a7) -> conv_bus3/9(i7)
  asiaa_adc5g/10(c1) -> conv_bus4/2(i1)
  asiaa_adc5g/11(c2) -> conv_bus4/3(i2)
  asiaa_adc5g/12(c3) -> conv_bus4/4(i3)
  asiaa_adc5g/13(c4) -> conv_bus4/5(i4)
  asiaa_adc5g/14(c5) -> conv_bus4/6(i5)
  asiaa_adc5g/15(c6) -> conv_bus4/7(i6)
  asiaa_adc5g/16(c7) -> conv_bus4/8(i7)
  [gain_adc] -> pipeline274/1
  asiaa_adc5g/9(c0) -> conv_bus4/1(i0)
  [sync_gen] -> pipeline130/1(d)
  conv_bus3/1(q0) -> pipeline115/1
  conv_bus3/2(q1) -> pipeline120/1
  conv_bus3/3(q2) -> pipeline125/1
  conv_bus3/4(q3) -> pipeline127/1
  conv_bus3/5(q4) -> pipeline128/1
  conv_bus3/6(q5) -> pipeline129/1
  conv_bus3/7(q6) -> pipeline114/1
  conv_bus3/8(q7) -> pipeline113/1
  bus_create5/1(bus_out) -> pipeline142/1(d)
  Constant16/1 -> adcsnap3/3(trig), adcsnap3/2(we)
  pipeline142/1(q) -> adcsnap3/1(din)
  conv_bus3/9(q8) -> [adc1_a_red]
  pipeline113/1 -> pipeline126/1(d), bus_create5/8(in8)
  pipeline114/1 -> pipeline124/1(d), bus_create5/7(in7)
  pipeline115/1 -> pipeline116/1(d), bus_create5/1(in1)
  pipeline120/1 -> pipeline117/1(d), bus_create5/2(in2)
  pipeline125/1 -> pipeline118/1(d), bus_create5/3(in3)
  pipeline127/1 -> pipeline121/1(d), bus_create5/4(in4)
  pipeline128/1 -> pipeline122/1(d), bus_create5/5(in5)
  pipeline129/1 -> pipeline123/1(d), bus_create5/6(in6)
  [sync_gen] -> pipeline147/1(d)
  conv_bus4/1(q0) -> pipeline131/1
  conv_bus4/2(q1) -> pipeline135/1
  conv_bus4/3(q2) -> pipeline140/1
  conv_bus4/4(q3) -> pipeline144/1
  conv_bus4/5(q4) -> pipeline145/1
  conv_bus4/6(q5) -> pipeline146/1
  conv_bus4/7(q6) -> pipeline107/1
  conv_bus4/8(q7) -> pipeline106/1
  bus_create7/1(bus_out) -> pipeline148/1(d)
  Constant15/1 -> adcsnap4/3(trig), adcsnap4/2(we)
  pipeline148/1(q) -> adcsnap4/1(din)
  pipeline106/1 -> pipeline141/1(d), bus_create7/8(in8)
  pipeline107/1 -> pipeline139/1(d), bus_create7/7(in7)
  pipeline131/1 -> pipeline132/1(d), bus_create7/1(in1)
  pipeline135/1 -> pipeline133/1(d), bus_create7/2(in2)
  pipeline140/1 -> pipeline134/1(d), bus_create7/3(in3)
  pipeline144/1 -> pipeline136/1(d), bus_create7/4(in4)
  pipeline145/1 -> pipeline137/1(d), bus_create7/5(in5)
  pipeline146/1 -> pipeline138/1(d), bus_create7/6(in6)
  Delay140/1 -> [fft2_sync], Delay141/1
  Delay139/1 -> [fft2_ch0], power12/1
  Black Box8/6 -> Terminator20/1
  Black Box8/1 -> Delay140/1
  Delay142/1 -> [fft2_ch1], power13/1
  Delay143/1 -> power14/1, [fft2_ch2]
  Delay144/1 -> [fft2_ch3], power15/1
  Black Box8/2 -> Delay139/1
  Black Box8/3 -> Delay142/1
  Delay141/1 -> Delay149/1
  power15/1 -> Delay152/1
  power13/1 -> Delay150/1
  power12/1 -> Delay148/1
  power14/1 -> Delay151/1
  Delay147/1 -> acc_cntrl6/2(sync)
  [acc_len] -> pipeline112/1
  [cnt_rst] -> pipeline255/1
  Delay153/1 -> pipeline156/1(d)
  pipeline167/1(q) -> simple_bram_vacc12/1(new_acc)
  pipeline163/1(q) -> simple_bram_vacc12/2(din)
  pipeline166/1(q) -> pipeline154/1(d)
  acc_cntrl6/1(new_acc) -> pipeline177/1(d)
  pipeline156/1(q) -> pipeline173/1(d)
  simple_bram_vacc12/1(dout) -> pipeline211/1(d)
  simple_bram_vacc12/2(valid) -> pipeline212/1(d)
  pipeline157/1(q) -> simple_bram_vacc9/1(new_acc)
  pipeline155/1(q) -> simple_bram_vacc9/2(din)
  simple_bram_vacc9/1(dout) -> pipeline213/1(d)
  simple_bram_vacc9/2(valid) -> pipeline149/1(d)
  pipeline161/1(q) -> simple_bram_vacc11/1(new_acc)
  pipeline160/1(q) -> simple_bram_vacc11/2(din)
  simple_bram_vacc11/1(dout) -> pipeline150/1(d)
  simple_bram_vacc11/2(valid) -> pipeline102/1(d)
  pipeline159/1(q) -> simple_bram_vacc10/1(new_acc)
  pipeline158/1(q) -> simple_bram_vacc10/2(din)
  simple_bram_vacc10/1(dout) -> pipeline152/1(d)
  simple_bram_vacc10/2(valid) -> pipeline153/1(d)
  Delay154/1 -> pipeline162/1(d)
  pipeline162/1(q) -> pipeline174/1(d)
  Delay145/1 -> pipeline164/1(d)
  pipeline164/1(q) -> pipeline175/1(d)
  Delay146/1 -> pipeline165/1(d)
  pipeline165/1(q) -> pipeline176/1(d)
  pipeline176/1(q) -> pipeline158/1(d)
  pipeline173/1(q) -> pipeline163/1(d)
  pipeline175/1(q) -> pipeline160/1(d)
  pipeline174/1(q) -> pipeline155/1(d)
  pipeline177/1(q) -> pipeline166/1(d), pipeline159/1(d), pipeline161/1(d), pipeline157/1(d), pipeline167/1(d)
  Delay157/1 -> Delay134/1
  power16/1 -> Delay138/1
  power10/1 -> Delay136/1
  power9/1 -> Delay135/1
  power11/1 -> Delay137/1
  [acc_len] -> pipeline256/1
  [cnt_rst] -> pipeline257/1
  pipeline195/1(q) -> simple_bram_vacc15/1(new_acc)
  pipeline191/1(q) -> simple_bram_vacc15/2(din)
  pipeline194/1(q) -> pipeline202/1(d)
  acc_cntrl7/1(new_acc) -> pipeline200/1(d)
  pipeline184/1(q) -> pipeline196/1(d)
  simple_bram_vacc15/1(dout) -> pipeline203/1(d)
  simple_bram_vacc15/2(valid) -> pipeline204/1(d)
  pipeline185/1(q) -> simple_bram_vacc8/1(new_acc)
  pipeline183/1(q) -> simple_bram_vacc8/2(din)
  simple_bram_vacc8/1(dout) -> pipeline205/1(d)
  simple_bram_vacc8/2(valid) -> pipeline206/1(d)
  pipeline189/1(q) -> simple_bram_vacc14/1(new_acc)
  pipeline188/1(q) -> simple_bram_vacc14/2(din)
  simple_bram_vacc14/1(dout) -> pipeline207/1(d)
  simple_bram_vacc14/2(valid) -> pipeline104/1(d)
  pipeline187/1(q) -> simple_bram_vacc13/1(new_acc)
  pipeline186/1(q) -> simple_bram_vacc13/2(din)
  simple_bram_vacc13/1(dout) -> pipeline209/1(d)
  simple_bram_vacc13/2(valid) -> pipeline210/1(d)
  pipeline190/1(q) -> pipeline197/1(d)
  pipeline192/1(q) -> pipeline198/1(d)
  pipeline193/1(q) -> pipeline199/1(d)
  pipeline199/1(q) -> pipeline186/1(d)
  pipeline196/1(q) -> pipeline191/1(d)
  pipeline198/1(q) -> pipeline188/1(d)
  pipeline197/1(q) -> pipeline183/1(d)
  pipeline200/1(q) -> pipeline194/1(d), pipeline189/1(d), pipeline187/1(d), pipeline185/1(d), pipeline195/1(d)
  Delay135/1 -> Shift45/1
  Delay136/1 -> Shift46/1
  Delay137/1 -> Shift47/1
  Delay138/1 -> Shift48/1
  pipeline202/1(q) -> Counter17/1
  pipeline203/1(q) -> Reinterpret12/1
  pipeline205/1(q) -> Reinterpret17/1
  pipeline207/1(q) -> Reinterpret18/1
  pipeline209/1(q) -> Reinterpret11/1
  pipeline211/1(q) -> Reinterpret13/1
  pipeline213/1(q) -> Reinterpret14/1
  pipeline150/1(q) -> Reinterpret15/1
  pipeline152/1(q) -> Reinterpret16/1
  pipeline154/1(q) -> Counter16/1
  Delay60/1 -> power7/1, [fft0_ch3]
  Delay59/1 -> power6/1, [fft0_ch2]
  Delay58/1 -> power5/1, [fft0_ch1]
  Delay35/1 -> power4/1, [fft0_ch0]
  Delay37/1 -> [fft0_sync], Delay57/1
  Black Box8/5 -> Delay144/1
  Black Box8/4 -> Delay143/1
  Black Box/3 -> Subsystem/1(data)
  Black Box/2 -> Convert16/1
  Convert16/1 -> Subsystem/2(en)
  gpio3/1 -> Black Box/4
  gps_ctrl/1(in_reg) -> Slice14/1, Slice13/1, Slice5/1
  Slice5/1 -> Convert17/1, Black Box/1
  Slice13/1 -> Black Box/2
  Slice14/1 -> Black Box/3
  gpio6/1 -> Delay78/1
  Black Box/5 -> gpio4/1
  Black Box/1 -> Terminator/1
  Black Box/4 -> Terminator4/1
  Convert17/1 -> Subsystem/3(rst)
  gps_ddmmyy/1(in_reg) -> Subsystem/5(ddmmyy)
  Subsystem/1(secs) -> Concat1/2, sec/1(out_reg)
  Subsystem/3(pps_debug) -> gpio5/1
  Subsystem/2(subsec) -> Concat1/3
  Concat1/1 -> [time]
  Delay78/1 -> Subsystem/4(pps)
  Subsystem1/1(Out1) -> Concat1/1
  Counter4/1 -> Slice8/1, Slice7/1, Slice6/1
  Slice6/1 -> Logical1/2
  Slice7/1 -> Logical1/3
  Subsystem3/1(Out1) -> pipeline53/1
  [gain] -> Mult5/2
  Mult5/1 -> pipeline15/1(d)
  pipeline49/1(q) -> pipeline16/1(d)
  pipeline30/1 -> Delay/1
  Slice8/1 -> Logical1/1
  Delay/1 -> Delay5/1
  Delay1/1 -> Delay9/1
  Convert2/1 -> Delay2/1
  pipeline50/1(q) -> pipeline13/1(d)
  pipeline94/1 -> Delay1/1
  pipeline53/1 -> Shift32/1
  Logical1/1 -> pipeline94/1
  Delay2/1 -> Mult5/1
  Delay5/1 -> pipeline50/1(d)
  Delay9/1 -> pipeline49/1(d)
  pipeline13/1(q) -> pipeline17/1(d)
  pipeline15/1(q) -> pipeline18/1(d)
  pipeline16/1(q) -> pipeline19/1(d)
  pipeline17/1(q) -> sync_tree2/1(In1)
  pipeline18/1(q) -> m0_tree2/1(In1)
  pipeline19/1(q) -> m0_en1/1(In1)
  [cnt_rst] -> pipeline269/1, pipeline270/1
  pipeline511/1 -> bus_create10/1(in1)
  pipeline664/1 -> bus_create10/2(in2)
  pipeline546/1 -> bus_create10/3(in3)
  pipeline577/1 -> bus_create10/4(in4)
  pipeline565/1 -> edge_detect11/1, pipeline566/1
  pipeline566/1 -> Logical9/2
  geth_pack/1(dout) -> ten_Gbe_v2/2(tx_data)
  geth_pack/2(dout_valid) -> ten_Gbe_v2/3(tx_valid)
  geth_pack/3(eof) -> ten_Gbe_v2/6(tx_end_of_frame)
  ten_Gbe_v2/12(rx_overrun) -> Delay159/1
  Delay159/1 -> ten_Gbe_v2/8(rx_overrun_ack)
  ten_Gbe_v2/3(led_tx) -> gpio7/1
  [addr_ten_g] -> ten_Gbe_v2/4(tx_dest_ip)
  [port_ten_g] -> Slice15/1
  Slice15/1 -> ten_Gbe_v2/5(tx_dest_port)
  Constant110/1 -> ten_Gbe_v2/7(rx_ack)
  ten_Gbe_v2/4(tx_afull) -> Terminator98/1
  ten_Gbe_v2/5(tx_overflow) -> Terminator101/1
  ten_Gbe_v2/6(rx_data) -> Terminator102/1
  ten_Gbe_v2/7(rx_valid) -> Terminator103/1
  ten_Gbe_v2/8(rx_source_ip) -> Terminator105/1
  ten_Gbe_v2/9(rx_source_port) -> Terminator106/1
  ten_Gbe_v2/10(rx_end_of_frame) -> Terminator107/1
  ten_Gbe_v2/11(rx_bad_frame) -> Terminator108/1
  ten_Gbe_v2/13(rx_dest_ip) -> Terminator109/1
  ten_Gbe_v2/14(rx_dest_port) -> Terminator99/1
  ten_Gbe_v2/2(led_rx) -> Terminator100/1
  bus_create10/1(bus_out) -> pipeline567/1
  [cnt_rst] -> pipeline271/1
  edge_detect11/1 -> Mux4/1, Register11/1, Register11/3, Logical9/1
  [cnt_rst] -> pipeline268/1
  pipeline567/1 -> Mux4/2
  Mux4/1 -> geth_pack/2(din)
  Register11/1 -> Logical25/2
  Logical9/1 -> Logical25/1
  Logical25/1 -> geth_pack/3(data_en)
  [time] -> Mux4/3
  power/1 -> pipeline348/1(d)
  power17/1 -> pipeline345/1(d)
  power18/1 -> pipeline346/1(d)
  power19/1 -> pipeline347/1(d)
  pipeline182/1(q) -> pipeline351/1(d)
  complex_convert/1(out) -> concat_order/1(ch0), power/1
  complex_convert1/1(out) -> concat_order/2(ch1), power17/1
  complex_convert2/1(out) -> concat_order/3(ch2), power18/1
  complex_convert3/1(out) -> concat_order/4(ch3), power19/1
  pipeline201/1(q) -> pipeline182/1(d), Black Box5/1
  adder_tree1/1(sync_out) -> Counter4/1, pipeline30/1
  adder_tree1/2(dout) -> Subsystem3/1(In1)
  pipeline347/1(q) -> Delay163/1
  pipeline345/1(q) -> Delay166/1
  Delay164/1 -> acc_cntrl8/2(sync)
  [acc_len] -> pipeline266/1
  [cnt_rst] -> pipeline267/1
  Delay165/1 -> pipeline221/1(d)
  pipeline232/1(q) -> simple_bram_vacc19/1(new_acc)
  pipeline228/1(q) -> simple_bram_vacc19/2(din)
  pipeline231/1(q) -> pipeline219/1(d)
  acc_cntrl8/1(new_acc) -> pipeline237/1(d)
  pipeline221/1(q) -> pipeline233/1(d)
  simple_bram_vacc19/1(dout) -> pipeline240/1(d)
  beam0/1(data_out) -> Terminator27/1
  simple_bram_vacc19/2(valid) -> pipeline241/1(d)
  pipeline222/1(q) -> simple_bram_vacc16/1(new_acc)
  pipeline220/1(q) -> simple_bram_vacc16/2(din)
  simple_bram_vacc16/1(dout) -> pipeline242/1(d)
  beam1/1(data_out) -> Terminator24/1
  simple_bram_vacc16/2(valid) -> pipeline214/1(d)
  pipeline226/1(q) -> simple_bram_vacc18/1(new_acc)
  pipeline225/1(q) -> simple_bram_vacc18/2(din)
  simple_bram_vacc18/1(dout) -> pipeline215/1(d)
  beam2/1(data_out) -> Terminator26/1
  simple_bram_vacc18/2(valid) -> pipeline216/1(d)
  pipeline224/1(q) -> simple_bram_vacc17/1(new_acc)
  pipeline223/1(q) -> simple_bram_vacc17/2(din)
  simple_bram_vacc17/1(dout) -> pipeline217/1(d)
  beam3/1(data_out) -> Terminator25/1
  simple_bram_vacc17/2(valid) -> pipeline218/1(d)
  Counter18/1 -> beam0/1(addr), beam1/1(addr), beam2/1(addr), beam3/1(addr)
  Delay166/1 -> pipeline227/1(d)
  pipeline227/1(q) -> pipeline234/1(d)
  Delay162/1 -> pipeline229/1(d)
  pipeline229/1(q) -> pipeline235/1(d)
  Delay163/1 -> pipeline230/1(d)
  pipeline230/1(q) -> pipeline236/1(d)
  pipeline351/1(q) -> Delay164/1
  pipeline348/1(q) -> Delay165/1
  pipeline346/1(q) -> Delay162/1
  pipeline236/1(q) -> pipeline223/1(d)
  pipeline233/1(q) -> pipeline228/1(d)
  pipeline235/1(q) -> pipeline225/1(d)
  pipeline234/1(q) -> pipeline220/1(d)
  pipeline237/1(q) -> pipeline231/1(d), pipeline224/1(d), pipeline226/1(d), pipeline222/1(d), pipeline232/1(d)
  Reinterpret19/1 -> beam0/2(data_in), pipeline248/1(d)
  Reinterpret20/1 -> beam1/2(data_in), pipeline246/1(d)
  Reinterpret21/1 -> pipeline244/1(d), beam2/2(data_in)
  Reinterpret22/1 -> pipeline243/1(d), beam3/2(data_in)
  pipeline239/1(q) -> pipeline238/1
  pipeline240/1(q) -> Reinterpret19/1
  pipeline241/1(q) -> beam0/3(we), Counter18/2
  pipeline242/1(q) -> Reinterpret20/1
  pipeline214/1(q) -> beam1/3(we)
  pipeline216/1(q) -> beam2/3(we)
  pipeline215/1(q) -> Reinterpret21/1
  pipeline217/1(q) -> Reinterpret22/1
  pipeline218/1(q) -> pipeline239/1(d), beam3/3(we)
  pipeline219/1(q) -> Counter18/1
  pipeline243/1(q) -> pipeline87/1
  pipeline244/1(q) -> pipeline245/1
  pipeline246/1(q) -> pipeline247/1
  pipeline248/1(q) -> pipeline249/1
  pipeline249/1 -> pipeline511/1
  pipeline247/1 -> pipeline664/1
  pipeline245/1 -> pipeline546/1
  pipeline87/1 -> pipeline577/1
  pipeline238/1 -> pipeline565/1
  pipeline250/1(q) -> pipeline201/1(d)
  pipeline251/1(q) -> complex_convert/1(in)
  pipeline252/1(q) -> complex_convert1/1(in)
  pipeline253/1(q) -> complex_convert2/1(in)
  pipeline254/1(q) -> complex_convert3/1(in)
  [acc_len0] -> pipeline259/1
  [cnt_rst] -> pipeline258/1
  [sd0] -> acc_cntrl2/2(sync)
  [m0d0] -> Delay26/1
  [m0e0] -> Delay27/1
  Delay26/1 -> Delay28/1
  acc_cntrl2/1(new_acc) -> Delay29/1
  Delay27/1 -> Delay30/1
  Delay29/1 -> pipeline9/1(d), simple_bram_vacc/1(new_acc)
  Delay30/1 -> simple_bram_vacc/3(val_in)
  Counter2/1 -> ACC0/1(addr)
  ACC0/1(data_out) -> Terminator22/1
  simple_bram_vacc/2(valid) -> pipeline/1
  simple_bram_vacc/1(dout) -> pipeline1/1
  pipeline1/1 -> Black Box1/2, Convert/1
  Counter1/1 -> small_spec2/1(addr)
  pipeline3/1(q) -> Reinterpret1/1
  pipeline4/1(q) -> Counter1/1
  pipeline7/1(q) -> small_spec2/3(we), Counter1/2
  Reinterpret1/1 -> small_spec2/2(data_in)
  pipeline8/1 -> pipeline4/1(d)
  Convert/1 -> pipeline3/1(d)
  pipeline9/1(q) -> pipeline8/1
  Delay28/1 -> simple_bram_vacc/2(din)
  pipeline/1 -> Black Box1/3, pipeline7/1(d)
  [acc_len2] -> pipeline262/1
  [cnt_rst] -> pipeline263/1
  [sd1] -> acc_cntrl1/2(sync)
  [m0d1] -> Delay19/1
  [m0e1] -> Delay20/1
  Delay19/1 -> Delay21/1
  acc_cntrl1/1(new_acc) -> Delay22/1
  Delay20/1 -> Delay24/1
  Delay22/1 -> simple_bram_vacc2/1(new_acc)
  Delay24/1 -> simple_bram_vacc2/3(val_in)
  Counter9/1 -> ACC2/1(addr)
  ACC2/1(data_out) -> Terminator1/1
  simple_bram_vacc2/2(valid) -> pipeline20/1
  simple_bram_vacc2/1(dout) -> pipeline21/1
  pipeline21/1 -> Black Box3/2
  Delay21/1 -> simple_bram_vacc2/2(din)
  pipeline20/1 -> Black Box3/3
  Black Box3/6 -> Convert24/1
  [acc_len3] -> pipeline264/1
  [cnt_rst] -> pipeline265/1
  [sd3] -> acc_cntrl4/2(sync)
  [m0d3] -> Delay40/1
  [m0e3] -> Delay41/1
  Delay40/1 -> Delay42/1
  acc_cntrl4/1(new_acc) -> Delay43/1
  Delay41/1 -> Delay45/1
  Delay43/1 -> simple_bram_vacc3/1(new_acc)
  Delay45/1 -> simple_bram_vacc3/3(val_in)
  Counter12/1 -> ACC3/1(addr)
  ACC3/1(data_out) -> Terminator2/1
  simple_bram_vacc3/2(valid) -> pipeline24/1
  simple_bram_vacc3/1(dout) -> pipeline25/1
  pipeline25/1 -> Black Box4/2
  Delay42/1 -> simple_bram_vacc3/2(din)
  [frb_detector_1] -> pipeline109/1
  [frb_detector_0] -> pipeline108/1
  pipeline111/1 -> Concat10/1, Logical12/4
  pipeline108/1 -> Concat10/4, Logical12/1
  pipeline109/1 -> Concat10/3, Logical12/2
  pipeline110/1 -> Concat10/2, Logical12/3
  [frb_detector_3] -> pipeline111/1
  [frb_detector_2] -> pipeline110/1
  Logical12/1 -> pipeline119/1
  pipeline119/1 -> Register3/1, Register3/3
  Register3/1 -> [detection]
  [rst_detect] -> Register3/2
  [acc_len1] -> pipeline260/1
  [cnt_rst] -> pipeline261/1
  [sd2] -> acc_cntrl5/2(sync)
  [m0d2] -> Delay54/1
  [m0e2] -> Delay55/1
  Delay54/1 -> Delay56/1
  acc_cntrl5/1(new_acc) -> Delay74/1
  Delay55/1 -> Delay76/1
  Delay74/1 -> simple_bram_vacc4/1(new_acc)
  Delay76/1 -> simple_bram_vacc4/3(val_in)
  Counter14/1 -> ACC1/1(addr)
  ACC1/1(data_out) -> Terminator3/1
  simple_bram_vacc4/2(valid) -> pipeline35/1
  simple_bram_vacc4/1(dout) -> pipeline45/1
  pipeline45/1 -> Black Box2/2
  Delay56/1 -> simple_bram_vacc4/2(din)
  pipeline35/1 -> Black Box2/3
  Convert15/1 -> frb_detector/1(out_reg)
  Black Box1/6 -> Convert23/1
  Black Box1/3 -> Terminator30/1
  Black Box1/4 -> Terminator31/1
  Black Box2/6 -> Convert22/1
  pipeline24/1 -> Black Box4/3
  Black Box4/6 -> Convert21/1
  Black Box2/1 -> Terminator32/1
  Black Box2/2 -> Terminator33/1
  Black Box2/3 -> Terminator34/1
  Black Box2/4 -> Terminator35/1
  Black Box3/1 -> Terminator36/1
  Black Box3/2 -> Terminator37/1
  Black Box3/3 -> Terminator38/1
  Black Box3/4 -> Terminator39/1
  Black Box4/1 -> Terminator40/1
  Black Box4/2 -> Terminator41/1
  Black Box4/3 -> Terminator42/1
  Black Box4/4 -> Terminator47/1
  Black Box2/5 -> Reinterpret6/1, ACC1/2(data_in)
  Black Box3/5 -> Reinterpret25/1, ACC2/2(data_in)
  [cnt_rst] -> Black Box1/1
  [cnt_rst] -> Black Box2/1
  [cnt_rst] -> Black Box3/1
  [cnt_rst] -> Black Box4/1
  Black Box4/5 -> Reinterpret27/1, ACC3/2(data_in)
  [rst] -> pipeline421/1
  [rst] -> pipeline422/1
  [gbe_data] -> pipeline423/1
  [gbe_valid] -> pipeline424/1
  [gbe_eof] -> pipeline430/1
  Delay91/1 -> pipeline428/1
  one_GbE/1 -> Terminator59/1
  one_GbE/2 -> Terminator60/1
  one_GbE/3 -> Terminator61/1
  one_GbE/4 -> Terminator53/1
  one_GbE/5 -> Terminator54/1
  one_GbE/6 -> Terminator55/1
  one_GbE/7 -> Terminator56/1
  one_GbE/8 -> Terminator57/1
  one_GbE/9 -> Terminator58/1
  one_GbE/10 -> Terminator51/1
  one_GbE/11 -> Terminator52/1
  Concat/1 -> pipeline406/1(d)
  ring/1(dout) -> pipeline403/1
  ring/2(eof) -> pipeline404/1
  ring/3(val) -> pipeline405/1
  pipeline407/1 -> Concat/1
  pipeline408/1 -> Concat/2
  pipeline409/1 -> Concat/3
  pipeline406/1(q) -> ring/2(data_in)
  [adc0_a_red] -> pipeline407/1
  [adc0_c_red] -> pipeline408/1
  [adc1_a_red] -> pipeline409/1
  [port_one_g] -> Delay92/1
  [addr_one_g] -> Delay91/1
  control1/1(in_reg) -> Slice12/1, Slice11/1, Slice10/1
  Slice10/1 -> Delay47/1
  Slice11/1 -> Delay49/1
  Delay47/1 -> [write]
  Delay49/1 -> [rst]
  Slice12/1 -> Delay50/1
  Delay50/1 -> [allow_detect]
  [detection] -> Delay93/1
  [write] -> Logical24/2
  Logical23/1 -> Logical24/1
  [allow_detect] -> Inverter3/1
  Logical24/1 -> gpio1/1, ring/1(write_en)
  Inverter3/1 -> Logical23/1
  pipeline403/1 -> [gbe_data]
  pipeline404/1 -> [gbe_eof]
  pipeline405/1 -> [gbe_valid]
  Delay93/1 -> Logical23/2
  pipeline421/1 -> one_GbE/1
  pipeline422/1 -> one_GbE/2
  pipeline423/1 -> one_GbE/3
  pipeline424/1 -> one_GbE/4
  pipeline428/1 -> one_GbE/5
  pipeline429/1 -> one_GbE/6
  pipeline430/1 -> one_GbE/7
  Delay92/1 -> pipeline429/1
  Constant105/1 -> one_GbE/8
  pipeline12/1 -> acc_cntrl11/3(rst)
  pipeline22/1 -> acc_cntrl11/1(acc_len)
  pipeline26/1 -> acc_cntrl3/1(acc_len)
  pipeline51/1 -> acc_cntrl3/3(rst)
  pipeline112/1 -> acc_cntrl6/1(acc_len)
  pipeline255/1 -> acc_cntrl6/3(rst)
  pipeline256/1 -> acc_cntrl7/1(acc_len)
  pipeline257/1 -> acc_cntrl7/3(rst)
  pipeline258/1 -> acc_cntrl2/3(rst)
  pipeline259/1 -> acc_cntrl2/1(acc_len)
  pipeline260/1 -> acc_cntrl5/1(acc_len)
  pipeline261/1 -> acc_cntrl5/3(rst)
  pipeline262/1 -> acc_cntrl1/1(acc_len)
  pipeline263/1 -> acc_cntrl1/3(rst)
  pipeline264/1 -> acc_cntrl4/1(acc_len)
  pipeline265/1 -> acc_cntrl4/3(rst)
  pipeline266/1 -> acc_cntrl8/1(acc_len)
  pipeline267/1 -> acc_cntrl8/3(rst)
  pipeline268/1 -> Register11/2
  pipeline269/1 -> geth_pack/1(rst)
  pipeline270/1 -> ten_Gbe_v2/9(debug_rst)
  pipeline271/1 -> ten_Gbe_v2/1(rst)
  pipeline272/1 -> conv_bus1/1(gain)
  pipeline273/1 -> conv_bus2/1(gain)
  pipeline274/1 -> conv_bus3/1(gain)
  Shift32/1 -> Reinterpret/1
  Reinterpret/1 -> Convert2/1
  Register9/1 -> [frb_detector_0]
  [rst_detect] -> Register9/2
  Reinterpret5/1 -> Relational12/1, Convert30/1
  Counter8/1 -> var0/1(addr), avg0/1(addr)
  Convert29/1 -> Reinterpret23/1
  Reinterpret23/1 -> var0/2(data_in)
  Convert31/1 -> Delay16/1, Reinterpret2/1
  Delay4/1 -> var0/3(we), Counter8/1, Delay3/1, avg0/3(we)
  Convert30/1 -> mov_var2/1(din)
  Convert28/1 -> Mult1/2
  Mult1/1 -> AddSub1/1
  Delay16/1 -> AddSub1/2
  Convert23/1 -> ACC0/3(we), Counter2/1, Delay13/1
  mov_var2/2(mov_var) -> Convert28/1, Convert29/1
  Delay13/1 -> mov_var2/2(din_valid)
  mov_var2/1(mov_avg) -> Convert31/1
  mov_var2/3(dout_valid) -> Delay4/1
  [rst_var] -> mov_var2/3(rst)
  [theta0] -> Mult1/1
  Black Box1/5 -> ACC0/2(data_in), Reinterpret5/1
  Counter10/1 -> thresh0/1(addr)
  Delay3/1 -> Delay10/1
  Black Box1/1 -> Terminator28/1
  Black Box1/2 -> Terminator29/1
  Register10/1 -> [frb_detector_1]
  [rst_detect] -> Register10/2
  Reinterpret6/1 -> Relational13/1, Convert26/1
  Convert27/1 -> Delay18/1
  Delay25/1 -> Delay23/1
  Convert26/1 -> mov_var1/1(din)
  Convert1/1 -> Mult2/2
  Mult2/1 -> AddSub2/1
  Delay18/1 -> AddSub2/2
  Convert22/1 -> Counter14/1, ACC1/3(we), Delay15/1
  mov_var1/2(mov_var) -> Convert1/1
  Delay15/1 -> mov_var1/2(din_valid)
  mov_var1/1(mov_avg) -> Convert27/1
  mov_var1/3(dout_valid) -> Delay25/1
  [rst_var] -> mov_var1/3(rst)
  [theta1] -> Mult2/1
  Counter6/1 -> thresh1/1(addr)
  Delay23/1 -> Delay11/1
  Register4/1 -> [frb_detector_2]
  [rst_detect] -> Register4/2
  Reinterpret25/1 -> Relational6/1, Convert18/1
  Convert19/1 -> Delay32/1
  Delay36/1 -> Delay34/1
  Convert18/1 -> mov_var3/1(din)
  Convert14/1 -> Mult3/2
  Mult3/1 -> AddSub3/1
  Delay32/1 -> AddSub3/2
  Convert24/1 -> Delay31/1, ACC2/3(we), Counter9/1
  mov_var3/2(mov_var) -> Convert14/1
  Delay31/1 -> mov_var3/2(din_valid)
  mov_var3/1(mov_avg) -> Convert19/1
  mov_var3/3(dout_valid) -> Delay36/1
  [rst_var] -> mov_var3/3(rst)
  [theta2] -> Mult3/1
  Counter15/1 -> thresh2/1(addr)
  Delay34/1 -> Delay12/1
  Register1/1 -> [frb_detector_3]
  [rst_detect] -> Register1/2
  Reinterpret27/1 -> Relational2/1, Convert13/1
  Convert20/1 -> Delay39/1
  Delay46/1 -> Delay44/1
  Convert13/1 -> mov_var4/1(din)
  Convert12/1 -> Mult4/2
  Mult4/1 -> AddSub4/1
  Delay39/1 -> AddSub4/2
  Convert21/1 -> Counter12/1, ACC3/3(we), Delay38/1
  mov_var4/2(mov_var) -> Convert12/1
  Delay38/1 -> mov_var4/2(din_valid)
  mov_var4/1(mov_avg) -> Convert20/1
  mov_var4/3(dout_valid) -> Delay46/1
  [rst_var] -> mov_var4/3(rst)
  [theta3] -> Mult4/1
  Counter19/1 -> thresh3/1(addr)
  Delay44/1 -> Delay51/1
  acc_dedisp/1(in_reg) -> dedisp_control/1(acc_dedisp)
  acc_number/1(in_reg) -> dedisp_control/2(acc_number)
  dedisp_control/1(acc0) -> [acc_len0]
  dedisp_control/2(acc1) -> [acc_len1]
  dedisp_control/3(acc2) -> [acc_len2]
  dedisp_control/4(acc3) -> [acc_len3]
  theta/1(in_reg) -> dedisp_control/3(theta_val)
  dedisp_control/5(theta0) -> [theta0]
  dedisp_control/6(theta1) -> [theta1]
  dedisp_control/7(theta2) -> [theta2]
  dedisp_control/8(theta3) -> [theta3]
  Convert3/1 -> Delay72/1
  Convert25/1 -> Delay73/1
  Delay48/1 -> Delay66/1
  Delay61/1 -> acc_cntrl7/2(sync)
  Delay82/1 -> pipeline193/1(d)
  Delay83/1 -> pipeline184/1(d)
  Delay84/1 -> pipeline190/1(d)
  Delay87/1 -> pipeline192/1(d)
  Counter22/1 -> spec1_1/1(addr), spec1_0/1(addr)
  simple_bram_vacc43/2(valid) -> pipeline29/1(d)
  simple_bram_vacc45/2(valid) -> pipeline100/1(d)
  Subsystem/4(debug) -> Terminator17/1
  pipeline275/1(q) -> Register5/1, Register6/1, Register7/1, Register8/1
  pipeline280/1 -> Relational11/1, Relational10/1, Relational9/1, Relational8/1
  Relational8/1 -> Register5/2
  Constant19/1 -> Relational8/2
  Constant12/1 -> Relational9/2
  Constant17/1 -> Relational10/2
  Constant18/1 -> Relational11/2
  Relational11/1 -> Register8/2
  Relational10/1 -> Register7/2
  Relational9/1 -> Register6/2
  pipeline278/1(q) -> [port_ten_g]
  pipeline276/1(q) -> [addr_one_g]
  pipeline277/1(q) -> [port_one_g]
  pipeline279/1(q) -> [addr_ten_g]
  Register5/1 -> pipeline276/1(d)
  Register6/1 -> pipeline277/1(d)
  Register7/1 -> pipeline279/1(d)
  Register8/1 -> pipeline278/1(d)
  ip_addr/1(in_reg) -> pipeline275/1(d)
  ip_sel/1(in_reg) -> Slice1/1
  Slice1/1 -> pipeline280/1
  [fft0_ch0] -> pipeline83/1(d)
  [fft1_ch0] -> pipeline84/1(d)
  [fft0_ch1] -> pipeline86/1(d)
  [fft1_ch1] -> pipeline168/1(d)
  [fft0_ch2] -> pipeline170/1(d)
  [fft1_ch2] -> pipeline171/1(d)
  [fft0_ch3] -> pipeline178/1(d)
  [fft1_ch3] -> pipeline179/1(d)
  [fft0_sync] -> pipeline181/1(d)
  pipeline83/1(q) -> complex_add/1(ff0_ch0)
  pipeline84/1(q) -> complex_add/2(fft1_ch0)
  pipeline86/1(q) -> complex_add/3(fft0_ch1)
  pipeline168/1(q) -> complex_add/4(fft1_ch1)
  pipeline170/1(q) -> complex_add/5(fft0_ch2)
  pipeline171/1(q) -> complex_add/6(fft1_ch2)
  pipeline178/1(q) -> complex_add/7(fft0_ch3)
  pipeline179/1(q) -> complex_add/8(fft1_ch3)
  pipeline181/1(q) -> complex_add/9(sync)
  complex_add/2(ch0) -> pipeline251/1(d)
  complex_add/3(ch1) -> pipeline252/1(d)
  complex_add/4(ch2) -> pipeline253/1(d)
  complex_add/5(ch3) -> pipeline254/1(d)
  complex_add/1(sync_out) -> pipeline250/1(d)
  spec2_0/1(data_out) -> Terminator45/1
  spec2_1/1(data_out) -> Terminator9/1
  pipeline90/1(q) -> Counter5/2
  Counter5/1 -> spec2_0/1(addr), spec2_1/1(addr)
  simple_bram_vacc6/2(valid) -> pipeline85/1(d)
  spec3_0/1(data_out) -> Terminator48/1
  spec3_1/1(data_out) -> Terminator15/1
  pipeline212/1(q) -> Counter16/2
  Counter16/1 -> spec3_0/1(addr), spec3_1/1(addr)
  spec4_0/1(data_out) -> Terminator49/1
  spec4_1/1(data_out) -> Terminator16/1
  pipeline204/1(q) -> Counter17/2
  Counter17/1 -> spec4_1/1(addr), spec4_0/1(addr)
  Shift33/1 -> Convert3/1
  Shift34/1 -> Convert25/1
  Shift35/1 -> Convert33/1
  Convert33/1 -> Delay64/1
  Convert32/1 -> Delay65/1
  Shift36/1 -> Convert32/1
  Reinterpret40/1 -> Concat2/1
  Reinterpret41/1 -> Concat2/2
  Concat2/1 -> spec1_0/2(data_in)
  pipeline29/1(q) -> spec1_0/3(we)
  pipeline28/1(q) -> spec1_1/3(we)
  Reinterpret42/1 -> Concat3/1
  Reinterpret43/1 -> Concat3/2
  Concat3/1 -> spec1_1/2(data_in)
  Delay106/1 -> Delay6/1
  Shift37/1 -> Convert35/1
  Shift38/1 -> Convert34/1
  Shift39/1 -> Convert37/1
  Shift40/1 -> Convert36/1
  Delay107/1 -> Shift37/1
  Delay108/1 -> Shift38/1
  Delay109/1 -> Shift39/1
  Delay110/1 -> Shift40/1
  Convert35/1 -> Delay104/1
  Convert34/1 -> Delay105/1
  Convert37/1 -> Delay101/1
  Convert36/1 -> Delay102/1
  Delay6/1 -> Delay103/1
  Delay149/1 -> Delay7/1
  Shift41/1 -> Convert39/1
  Shift42/1 -> Convert38/1
  Shift43/1 -> Convert41/1
  Shift44/1 -> Convert40/1
  Delay148/1 -> Shift41/1
  Delay150/1 -> Shift42/1
  Delay151/1 -> Shift43/1
  Delay152/1 -> Shift44/1
  Delay7/1 -> Delay147/1
  Convert39/1 -> Delay153/1
  Convert38/1 -> Delay154/1
  Convert41/1 -> Delay145/1
  Convert40/1 -> Delay146/1
  Delay134/1 -> Delay8/1
  Shift45/1 -> Convert43/1
  Shift46/1 -> Convert42/1
  Shift47/1 -> Convert45/1
  Shift48/1 -> Convert44/1
  Delay8/1 -> Delay61/1
  Convert43/1 -> Delay83/1
  Convert42/1 -> Delay84/1
  Convert45/1 -> Delay87/1
  Convert44/1 -> Delay82/1
  Reinterpret4/1 -> Concat4/1
  Reinterpret8/1 -> Concat4/2
  Concat4/1 -> spec2_0/2(data_in)
  pipeline92/1(q) -> spec2_0/3(we)
  Reinterpret9/1 -> Concat5/1
  Reinterpret10/1 -> Concat5/2
  Concat5/1 -> spec2_1/2(data_in)
  pipeline96/1(q) -> spec2_1/3(we)
  Reinterpret13/1 -> Concat6/1
  Reinterpret14/1 -> Concat6/2
  Concat6/1 -> spec3_0/2(data_in)
  pipeline149/1(q) -> spec3_0/3(we)
  Reinterpret15/1 -> Concat7/1
  Reinterpret16/1 -> Concat7/2
  Concat7/1 -> spec3_1/2(data_in)
  pipeline153/1(q) -> spec3_1/3(we)
  Reinterpret12/1 -> Concat8/1
  Reinterpret17/1 -> Concat8/2
  Concat8/1 -> spec4_0/2(data_in)
  pipeline206/1(q) -> spec4_0/3(we)
  Reinterpret18/1 -> Concat9/1
  Reinterpret11/1 -> Concat9/2
  Concat9/1 -> spec4_1/2(data_in)
  pipeline210/1(q) -> spec4_1/3(we)
  pipeline104/1(q) -> Terminator8/1
  pipeline102/1(q) -> Terminator10/1
  pipeline85/1(q) -> Terminator11/1
  pipeline100/1(q) -> Terminator13/1
  Slice2/1 -> pipeline151/1(d)
  pipeline151/1(q) -> [rst_var]
  pipeline5/1(q) -> Slice2/1, Slice3/1, Slice/1
  Reinterpret2/1 -> avg0/2(data_in)
  Reinterpret3/1 -> thresh0/2(data_in)
  thresh_offset/1(in_reg) -> dedisp_control/4(offset)
  dedisp_control/9(off0) -> [off0]
  dedisp_control/10(off1) -> [off1]
  dedisp_control/11(off2) -> [off2]
  dedisp_control/12(off3) -> [off3]
  AddSub1/1 -> AddSub5/2
  AddSub5/1 -> Reinterpret3/1, Relational12/2
  [off0] -> AddSub5/1
  Delay10/1 -> thresh0/3(we), Counter10/1
  Delay11/1 -> thresh1/3(we), Counter6/1
  AddSub2/1 -> AddSub6/2
  AddSub6/1 -> thresh1/2(data_in), Relational13/2
  [off1] -> AddSub6/1
  Delay12/1 -> thresh2/3(we), Counter15/1
  AddSub3/1 -> AddSub7/2
  AddSub7/1 -> Relational6/2, thresh2/2(data_in)
  [off2] -> AddSub7/1
  AddSub4/1 -> AddSub8/2
  AddSub8/1 -> Relational2/2, thresh3/2(data_in)
  Delay51/1 -> thresh3/3(we), Counter19/1
  [off3] -> AddSub8/1
  Concat10/1 -> Convert15/1
  pipeline39/1(q) -> Black Box6/8
  pipeline33/1(q) -> Black Box6/3
  pipeline38/1(q) -> Black Box6/7
  pipeline37/1(q) -> Black Box6/6
  pipeline36/1(q) -> Black Box6/5
  pipeline34/1(q) -> Black Box6/4
  pipeline40/1(q) -> Black Box6/9
  pipeline32/1(q) -> Black Box6/2
  pipeline41/1(q) -> Black Box6/1
  pipeline57/1(q) -> Black Box7/8
  pipeline44/1(q) -> Black Box7/3
  pipeline56/1(q) -> Black Box7/7
  pipeline55/1(q) -> Black Box7/6
  pipeline48/1(q) -> Black Box7/5
  pipeline46/1(q) -> Black Box7/4
  pipeline59/1(q) -> Black Box7/9
  pipeline43/1(q) -> Black Box7/2
  pipeline63/1(q) -> Black Box7/1
  pipeline130/1(q) -> Black Box8/1
  pipeline116/1(q) -> Black Box8/2
  pipeline117/1(q) -> Black Box8/3
  pipeline118/1(q) -> Black Box8/4
  pipeline121/1(q) -> Black Box8/5
  pipeline122/1(q) -> Black Box8/6
  pipeline123/1(q) -> Black Box8/7
  pipeline124/1(q) -> Black Box8/8
  pipeline126/1(q) -> Black Box8/9
  pipeline147/1(q) -> Black Box13/1
  pipeline132/1(q) -> Black Box13/2
  pipeline133/1(q) -> Black Box13/3
  pipeline134/1(q) -> Black Box13/4
  pipeline136/1(q) -> Black Box13/5
  pipeline137/1(q) -> Black Box13/6
  pipeline138/1(q) -> Black Box13/7
  pipeline139/1(q) -> Black Box13/8
  pipeline141/1(q) -> Black Box13/9
  Black Box13/1 -> Delay156/1
  Black Box13/2 -> Delay155/1
  Black Box13/3 -> Delay158/1
  Black Box13/4 -> Delay160/1
  Black Box13/5 -> Delay161/1
  Black Box13/6 -> Terminator19/1
  Subsystem2/1(syncout) -> [sync_beam]
  Subsystem2/2(dout0) -> [beam0]
  Subsystem2/3(dout1) -> [beam1]
  Subsystem2/4(dout2) -> [beam2]
  Subsystem2/5(dout3) -> [beam3]
  [gain_rfi] -> Subsystem2/1(gain)
  [fft3_sync] -> pipeline169/1
  [fft3_ch0] -> pipeline172/1
  [fft3_ch1] -> pipeline285/1
  [fft3_ch2] -> pipeline287/1
  [fft3_ch3] -> pipeline288/1
  pipeline169/1 -> pipeline289/1
  pipeline172/1 -> pipeline290/1
  pipeline285/1 -> pipeline291/1
  pipeline287/1 -> pipeline180/1
  pipeline288/1 -> pipeline208/1
  pipeline289/1 -> pipeline281/1
  pipeline290/1 -> pipeline282/1
  pipeline291/1 -> pipeline283/1
  pipeline180/1 -> pipeline284/1
  pipeline208/1 -> pipeline286/1
  pipeline281/1 -> pipeline292/1(d)
  pipeline282/1 -> pipeline293/1(d)
  pipeline283/1 -> pipeline294/1(d)
  pipeline284/1 -> pipeline295/1(d)
  pipeline286/1 -> pipeline296/1(d)
  Subsystem4/1(syncout) -> [sync_rfi]
  Subsystem4/2(Out1) -> [rfi0]
  Subsystem4/3(Out2) -> [rfi1]
  Subsystem4/4(Out3) -> [rfi2]
  Subsystem4/5(Out4) -> [rfi3]
  [gain_rfi] -> Subsystem4/1(gain)
  Delay156/1 -> Delay157/1, [fft3_sync]
  Delay155/1 -> power9/1, [fft3_ch0]
  Delay158/1 -> power10/1, [fft3_ch1]
  Delay160/1 -> power11/1, [fft3_ch2]
  Delay161/1 -> power16/1, [fft3_ch3]
  gain_rfi/1(in_reg) -> pipeline322/1(d)
  pipeline322/1(q) -> [gain_rfi]
  acc_len_rfi/1(in_reg) -> pipeline376/1(d)
  pipeline376/1(q) -> [acc_len_rfi]
  Constant/1 -> asiaa_adc5g/1(sim_a)
  Constant21/1 -> asiaa_adc5g/2(sim_c)
  Constant22/1 -> asiaa_adc5g/3(sim_sync)
  Constant23/1 -> asiaa_adc5g1/1(sim_a)
  Constant24/1 -> asiaa_adc5g1/2(sim_c)
  Constant25/1 -> asiaa_adc5g1/3(sim_sync)
  pipeline510/1(q) -> pipeline447/1(d)
  [cnt_rst] -> acc_cntrl13/3(rst)
  [acc_len_rfi] -> acc_cntrl13/1(acc_len)
  pipeline512/1(q) -> simple_bram_vacc_0c_4/2(din)
  pipeline496/1(q) -> simple_bram_vacc_0c_4/1(new_acc)
  pipeline498/1(q) -> simple_bram_vacc_0c_5/2(din)
  pipeline501/1(q) -> simple_bram_vacc_0c_5/1(new_acc)
  pipeline502/1(q) -> simple_bram_vacc_0c_20/2(din)
  pipeline505/1(q) -> simple_bram_vacc_0c_20/1(new_acc)
  pipeline506/1(q) -> simple_bram_vacc_0c_21/2(din)
  pipeline509/1(q) -> simple_bram_vacc_0c_21/1(new_acc)
  Delay212/1 -> pipeline512/1(d)
  Delay220/1 -> pipeline498/1(d)
  Delay222/1 -> pipeline502/1(d)
  Delay203/1 -> pipeline506/1(d)
  acc_cntrl13/1(new_acc) -> pipeline497/1(d), pipeline496/1(d), pipeline505/1(d), pipeline509/1(d), pipeline501/1(d)
  pipeline457/1(q) -> pipeline448/1(d)
  [cnt_rst] -> acc_cntrl14/3(rst)
  [acc_len_rfi] -> acc_cntrl14/1(acc_len)
  pipeline483/1(q) -> simple_bram_vacc_0a_1/2(din)
  pipeline489/1(q) -> simple_bram_vacc_0a_1/1(new_acc)
  pipeline491/1(q) -> simple_bram_vacc_0a_2/2(din)
  pipeline494/1(q) -> simple_bram_vacc_0a_2/1(new_acc)
  pipeline514/1(q) -> simple_bram_vacc_0a_3/2(din)
  pipeline518/1(q) -> simple_bram_vacc_0a_3/1(new_acc)
  pipeline519/1(q) -> simple_bram_vacc_0a_8/2(din)
  pipeline446/1(q) -> simple_bram_vacc_0a_8/1(new_acc)
  Delay225/1 -> pipeline483/1(d)
  Delay226/1 -> pipeline491/1(d)
  Delay227/1 -> pipeline514/1(d)
  Delay228/1 -> pipeline519/1(d)
  acc_cntrl14/1(new_acc) -> pipeline494/1(d), pipeline446/1(d), pipeline518/1(d), pipeline489/1(d), pipeline490/1(d)
  complex_conj4/1(z*) -> cmult4/2(b)
  Delay202/1 -> cmult4/1(a)
  complex_conj5/1(z*) -> cmult5/2(b)
  Delay230/1 -> cmult5/1(a)
  complex_conj6/1(z*) -> cmult6/2(b)
  Delay231/1 -> cmult6/1(a)
  complex_conj7/1(z*) -> cmult7/2(b)
  Delay232/1 -> cmult7/1(a)
  Delay213/1 -> pipeline510/1(d)
  Delay223/1 -> power38/1
  Delay224/1 -> power39/1
  Delay229/1 -> power40/1
  Delay236/1 -> power41/1
  Delay204/1 -> pipeline457/1(d)
  Delay205/1 -> power42/1
  Delay206/1 -> power43/1
  Delay207/1 -> power32/1
  Delay208/1 -> power33/1
  [beam0] -> Delay202/1
  [rfi0] -> complex_conj4/1(z)
  [beam1] -> Delay230/1
  [rfi1] -> complex_conj5/1(z)
  [beam2] -> Delay231/1
  [rfi2] -> complex_conj6/1(z)
  [beam3] -> Delay232/1
  [rfi3] -> complex_conj7/1(z)
  pipeline418/1(q) -> pipeline449/1(d)
  [cnt_rst] -> acc_cntrl15/3(rst)
  [acc_len_rfi] -> acc_cntrl15/1(acc_len)
  corr0/1(data_out) -> Terminator73/1
  Reinterpret100/1 -> corr0/2(data_in)
  pipeline410/1(q) -> simple_bram_vacc_0c_22/2(din)
  pipeline521/1(q) -> corr0/3(we), Counter23/2
  pipeline522/1(q) -> Counter23/1
  pipeline523/1(q) -> simple_bram_vacc_0c_22/1(new_acc)
  corr1/1(data_out) -> Terminator79/1
  Reinterpret71/1 -> corr1/2(data_in)
  pipeline525/1(q) -> simple_bram_vacc_0c_23/2(din)
  pipeline527/1(q) -> corr1/3(we)
  pipeline528/1(q) -> simple_bram_vacc_0c_23/1(new_acc)
  corr2/1(data_out) -> Terminator72/1
  Reinterpret88/1 -> corr2/2(data_in)
  pipeline377/1(q) -> simple_bram_vacc_0c_6/2(din)
  pipeline382/1(q) -> corr2/3(we)
  pipeline383/1(q) -> simple_bram_vacc_0c_6/1(new_acc)
  corr3/1(data_out) -> Terminator44/1
  Reinterpret99/1 -> corr3/2(data_in)
  pipeline385/1(q) -> simple_bram_vacc_0c_7/2(din)
  pipeline390/1(q) -> corr3/3(we)
  pipeline393/1(q) -> simple_bram_vacc_0c_7/1(new_acc)
  Delay210/1 -> pipeline410/1(d)
  Delay211/1 -> pipeline525/1(d)
  Delay214/1 -> pipeline377/1(d)
  Delay209/1 -> pipeline385/1(d)
  Counter23/1 -> corr3/1(addr), corr2/1(addr), corr1/1(addr), corr0/1(addr)
  Delay215/1 -> pipeline418/1(d)
  [beam0] -> Delay223/1
  [beam1] -> Delay224/1
  [beam2] -> Delay229/1
  [beam3] -> Delay236/1
  [sync_beam] -> Delay213/1
  [sync_rfi] -> Delay204/1
  [rfi0] -> Delay205/1
  [rfi1] -> Delay206/1
  [rfi2] -> Delay207/1
  [rfi3] -> Delay208/1
  [sync_beam] -> Delay215/1
  cmult4/1(ab) -> pipeline450/1(d)
  c_to_ri4/1 -> Delay210/1
  c_to_ri4/2 -> Delay211/1
  cmult5/1(ab) -> pipeline451/1(d)
  c_to_ri5/1 -> Delay214/1
  c_to_ri5/2 -> Delay209/1
  pipeline445/1(q) -> simple_bram_vacc_0c_18/2(din)
  pipeline420/1(q) -> simple_bram_vacc_0c_18/1(new_acc)
  pipeline426/1(q) -> simple_bram_vacc_0c_19/2(din)
  pipeline432/1(q) -> simple_bram_vacc_0c_19/1(new_acc)
  pipeline441/1(q) -> simple_bram_vacc_0c_16/2(din)
  pipeline442/1(q) -> simple_bram_vacc_0c_16/1(new_acc)
  pipeline443/1(q) -> simple_bram_vacc_0c_17/2(din)
  pipeline444/1(q) -> simple_bram_vacc_0c_17/1(new_acc)
  Delay217/1 -> pipeline445/1(d)
  Delay233/1 -> pipeline426/1(d)
  Delay218/1 -> pipeline441/1(d)
  Delay216/1 -> pipeline443/1(d)
  acc_cntrl15/1(new_acc) -> pipeline524/1(d), pipeline523/1(d), pipeline420/1(d), pipeline444/1(d), pipeline442/1(d), pipeline432/1(d), pipeline393/1(d), pipeline383/1(d), pipeline528/1(d)
  cmult6/1(ab) -> pipeline452/1(d)
  c_to_ri6/1 -> Delay217/1
  c_to_ri6/2 -> Delay233/1
  cmult7/1(ab) -> pipeline453/1(d)
  c_to_ri7/1 -> Delay218/1
  c_to_ri7/2 -> Delay216/1
  simple_bram_vacc_0c_22/1(dout) -> ri_to_c4/1
  simple_bram_vacc_0c_23/1(dout) -> ri_to_c4/2
  simple_bram_vacc_0c_6/1(dout) -> ri_to_c5/1
  simple_bram_vacc_0c_7/1(dout) -> ri_to_c5/2
  simple_bram_vacc_0c_18/1(dout) -> ri_to_c6/1
  simple_bram_vacc_0c_19/1(dout) -> ri_to_c6/2
  simple_bram_vacc_0c_16/1(dout) -> ri_to_c7/1
  simple_bram_vacc_0c_17/1(dout) -> ri_to_c7/2
  power38/1 -> Reinterpret78/1
  power39/1 -> Reinterpret79/1
  power40/1 -> Reinterpret80/1
  power41/1 -> Reinterpret81/1
  power32/1 -> Reinterpret85/1
  power33/1 -> Reinterpret86/1
  power43/1 -> Reinterpret84/1
  power42/1 -> Reinterpret83/1
  pipeline447/1(q) -> acc_cntrl13/2(sync)
  pipeline448/1(q) -> acc_cntrl14/2(sync)
  pipeline449/1(q) -> acc_cntrl15/2(sync)
  pipeline450/1(q) -> c_to_ri4/1
  pipeline451/1(q) -> c_to_ri5/1
  pipeline452/1(q) -> c_to_ri6/1
  pipeline453/1(q) -> c_to_ri7/1
  power34/1 -> Reinterpret87/1
  pipeline414/1(q) -> pipeline467/1(d)
  pipeline454/1(q) -> pipeline521/1(d)
  power35/1 -> Reinterpret89/1
  pipeline456/1(q) -> pipeline527/1(d)
  pipeline455/1(q) -> pipeline382/1(d)
  pipeline458/1(q) -> pipeline390/1(d)
  power36/1 -> Reinterpret90/1
  power37/1 -> Reinterpret91/1
  Subsystem6/2(ch0) -> Convert73/1
  Subsystem6/3(ch1) -> Convert74/1
  Subsystem6/4(ch2) -> Convert75/1
  Subsystem6/5(ch3) -> Convert76/1
  Subsystem6/1(sync_out) -> pipeline468/1(d)
  Subsystem6/6(valid_out) -> pipeline469/1(d)
  Reinterpret66/1 -> Convert47/1
  Reinterpret69/1 -> Convert48/1
  Reinterpret72/1 -> Convert50/1
  Reinterpret70/1 -> Convert49/1
  Reinterpret74/1 -> Convert52/1
  Reinterpret73/1 -> Convert51/1
  Reinterpret77/1 -> Convert54/1
  Reinterpret75/1 -> Convert53/1
  pipeline413/1(q) -> [corr0], Reinterpret100/1
  pipeline526/1(q) -> [corr1], Reinterpret71/1
  pipeline378/1(q) -> [corr2], Reinterpret88/1
  pipeline389/1(q) -> [corr3], Reinterpret99/1
  pipeline459/1(q) -> Delay212/1
  pipeline460/1(q) -> Delay220/1
  pipeline461/1(q) -> Delay222/1
  pipeline462/1(q) -> Delay203/1
  pipeline463/1(q) -> Delay225/1
  pipeline464/1(q) -> Delay226/1
  pipeline465/1(q) -> Delay227/1
  pipeline466/1(q) -> Delay228/1
  Reinterpret78/1 -> pipeline459/1(d)
  Reinterpret79/1 -> pipeline460/1(d)
  Reinterpret80/1 -> pipeline461/1(d)
  Reinterpret81/1 -> pipeline462/1(d)
  Reinterpret85/1 -> pipeline465/1(d)
  Reinterpret86/1 -> pipeline466/1(d)
  Reinterpret84/1 -> pipeline464/1(d)
  Reinterpret83/1 -> pipeline463/1(d)
  Reinterpret87/1 -> Convert72/1
  Reinterpret89/1 -> Convert71/1
  Reinterpret90/1 -> Convert60/1
  Reinterpret91/1 -> Convert59/1
  Convert59/1 -> pipeline389/1(d)
  Convert60/1 -> pipeline378/1(d)
  Convert71/1 -> pipeline526/1(d)
  Convert72/1 -> pipeline413/1(d)
  pipeline467/1(q) -> pipeline522/1(d)
  Convert73/1 -> pipeline473/1(d)
  Convert74/1 -> pipeline474/1(d)
  Convert75/1 -> pipeline475/1(d)
  Convert76/1 -> pipeline471/1(d)
  pipeline468/1(q) -> pipeline472/1(d)
  pipeline469/1(q) -> pipeline470/1(d)
  pipeline470/1(q) -> [mul_val]
  pipeline471/1(q) -> [mul3]
  pipeline472/1(q) -> [sync_mul]
  pipeline473/1(q) -> [mul0]
  pipeline474/1(q) -> [mul1]
  pipeline475/1(q) -> [mul2]
  mul0/1(data_out) -> Terminator82/1
  Reinterpret95/1 -> mul0/2(data_in)
  pipeline485/1(q) -> Reinterpret95/1
  pipeline476/1(q) -> mul0/3(we), Counter27/2
  pipeline477/1(q) -> Counter27/1
  mul1/1(data_out) -> Terminator78/1
  Reinterpret92/1 -> mul1/2(data_in)
  pipeline478/1(q) -> Reinterpret92/1
  pipeline479/1(q) -> mul1/3(we)
  mul2/1(data_out) -> Terminator80/1
  Reinterpret93/1 -> mul2/2(data_in)
  pipeline480/1(q) -> Reinterpret93/1
  pipeline481/1(q) -> mul2/3(we)
  mul3/1(data_out) -> Terminator81/1
  Reinterpret94/1 -> mul3/2(data_in)
  pipeline482/1(q) -> Reinterpret94/1
  pipeline484/1(q) -> mul3/3(we)
  Counter27/1 -> mul0/1(addr), mul1/1(addr), mul2/1(addr), mul3/1(addr)
  [sync_mul] -> pipeline477/1(d)
  [mul0] -> pipeline485/1(d)
  [mul1] -> pipeline478/1(d)
  [mul2] -> pipeline480/1(d)
  [mul3] -> pipeline482/1(d)
  [mul_val] -> pipeline476/1(d), pipeline479/1(d), pipeline481/1(d), pipeline484/1(d)
  [corr0] -> Black Box11/2
  [mul0] -> Black Box11/1
  [mul_val] -> Black Box11/3
  Black Box11/1 -> Reinterpret75/1
  Black Box11/2 -> Reinterpret77/1
  Black Box11/3 -> Convert61/1
  Convert77/1 -> Delay14/1
  Convert78/1 -> Delay173/1
  Convert69/1 -> Delay17/1
  Black Box10/1 -> Reinterpret73/1
  Black Box10/2 -> Reinterpret74/1
  Black Box10/3 -> Convert69/1
  [mul1] -> Black Box10/1
  [mul_val] -> Black Box10/3
  [corr1] -> Black Box10/2
  Black Box9/1 -> Reinterpret70/1
  [mul2] -> Black Box9/1
  Black Box9/2 -> Reinterpret72/1
  Black Box9/3 -> Convert78/1
  [mul_val] -> Black Box9/3
  [corr2] -> Black Box9/2
  Black Box12/1 -> Reinterpret66/1
  Black Box12/2 -> Reinterpret69/1
  Black Box12/3 -> Convert77/1
  [mul_val] -> Black Box12/3
  [mul3] -> Black Box12/1
  [corr3] -> Black Box12/2
  concat_order/1(Out1) -> Black Box5/2
  Black Box5/2 -> Slice17/1, Slice16/1, Slice9/1, Slice4/1
  Black Box5/1 -> Convert46/1
  Convert46/1 -> Subsystem2/2(sync), pipeline327/1(d)
  pipeline295/1(q) -> Subsystem4/5(In3)
  pipeline292/1(q) -> Subsystem4/2(sync)
  pipeline293/1(q) -> Subsystem4/3(In2)
  pipeline294/1(q) -> Subsystem4/4(In1)
  pipeline296/1(q) -> Subsystem4/6(In4)
  Counter/1 -> rfi/1(addr)
  "CORDIC 4.0 "/1 -> Relational5/1, Reinterpret7/1
  CORDIC 4.0 1/1 -> Relational7/1, Reinterpret24/1
  CORDIC 4.0 2/1 -> Relational14/1, Reinterpret26/1
  CORDIC 4.0 3/1 -> Relational15/1, Reinterpret28/1
  "CORDIC 4.0 "/2 -> Delay62/1, rfi/3(we), Counter/2
  Concat11/1 -> rfi/2(data_in)
  Reinterpret7/1 -> Concat11/1
  Reinterpret24/1 -> Concat11/2
  Reinterpret26/1 -> Concat11/3
  Reinterpret28/1 -> Concat11/4
  Delay33/1 -> Counter/1
  CORDIC 4.0 1/2 -> Terminator14/1
  CORDIC 4.0 2/2 -> Terminator18/1
  CORDIC 4.0 3/2 -> Terminator21/1
  [sync_mul] -> Delay33/1
  Convert47/1 -> Mux/2, Relational/2
  Relational/1 -> Mux/1
  Constant1/1 -> Relational/1
  Constant2/1 -> Mux/3
  Delay52/1 -> "CORDIC 4.0 "/2
  Convert48/1 -> Delay52/1
  Mux/1 -> "CORDIC 4.0 "/1
  Delay14/1 -> Delay133/1
  Delay133/1 -> "CORDIC 4.0 "/3
  Convert49/1 -> Mux1/2, Relational1/2
  Relational1/1 -> Mux1/1
  Constant3/1 -> Relational1/1
  Constant4/1 -> Mux1/3
  Delay167/1 -> CORDIC 4.0 1/2
  Convert50/1 -> Delay167/1
  Mux1/1 -> CORDIC 4.0 1/1
  Delay173/1 -> Delay168/1
  Delay168/1 -> CORDIC 4.0 1/3
  Convert51/1 -> Mux2/2, Relational3/2
  Relational3/1 -> Mux2/1
  Constant5/1 -> Relational3/1
  Constant7/1 -> Mux2/3
  Delay169/1 -> CORDIC 4.0 2/2
  Convert52/1 -> Delay169/1
  Mux2/1 -> CORDIC 4.0 2/1
  Delay17/1 -> Delay170/1
  Delay170/1 -> CORDIC 4.0 2/3
  Convert53/1 -> Mux3/2, Relational4/2
  Relational4/1 -> Mux3/1
  Constant8/1 -> Relational4/1
  Constant9/1 -> Mux3/3
  Delay171/1 -> CORDIC 4.0 3/2
  Convert54/1 -> Delay171/1
  Mux3/1 -> CORDIC 4.0 3/1
  Delay174/1 -> Delay172/1
  Delay172/1 -> CORDIC 4.0 3/3
  Convert61/1 -> Delay174/1
  rfi_flag/1(in_reg) -> pipeline2/1(d)
  pipeline2/1(q) -> Slice20/1, Slice19/1, Slice18/1
  Slice18/1 -> Convert56/1
  Slice19/1 -> Convert55/1
  Slice20/1 -> [flag_en]
  [flag_rfi] -> Black Box5/3
  [flag_num] -> Black Box5/4
  [flag_en] -> Black Box5/5
  Black Box7/6 -> Terminator5/1
  Black Box7/1 -> Delay86/1
  Black Box7/2 -> Delay85/1
  Black Box7/3 -> Delay94/1
  Black Box7/4 -> Delay95/1
  Black Box7/5 -> Delay96/1
  Convert55/1 -> [flag_num]
  Convert56/1 -> [flag_rfi]
  rfi_thresh/1(in_reg) -> Slice22/1, Slice21/1, Slice24/1, Slice23/1
  Slice21/1 -> pipeline23/1(d)
  Slice22/1 -> pipeline27/1(d)
  Slice23/1 -> pipeline52/1(d)
  Slice24/1 -> Reinterpret29/1
  pipeline23/1(q) -> [rfi_thresh_en]
  pipeline27/1(q) -> [rfi_count_en]
  pipeline297/1(q) -> [rfi_thresh]
  pipeline52/1(q) -> [rfi_count]
  Reinterpret29/1 -> pipeline297/1(d)
  [rfi_thresh_en] -> Register/2
  [rfi_thresh] -> Register/1
  Register/1 -> Delay53/1
  Delay53/1 -> Relational15/2, Relational14/2, Relational7/2, Relational5/2
  Relational5/1 -> Logical/1
  Relational7/1 -> Logical/2
  Relational14/1 -> Logical/3
  Relational15/1 -> Logical/4
  Delay62/1 -> Logical2/1
  Logical/1 -> Logical2/2
  Logical2/1 -> Register2/1, Register2/3
  Register2/1 -> Counter3/2, pipeline302/1(d)
  Counter3/1 -> Relational16/2
  Relational16/1 -> gpio2/1, Register2/2, Counter3/1
  Register12/1 -> Relational16/1
  [rfi_count] -> Register12/1
  [rfi_count_en] -> Register12/2
  Relational2/1 -> Logical3/2
  Inverter/1 -> Logical3/1
  pipeline302/1(q) -> [rfi_detection]
  Logical3/1 -> Register1/3, Register1/1
  [rfi_detection] -> Inverter/1
  Relational6/1 -> Logical4/2
  Inverter1/1 -> Logical4/1
  [rfi_detection] -> Inverter1/1
  Logical4/1 -> Register4/3, Register4/1
  Relational13/1 -> Logical5/2
  Inverter2/1 -> Logical5/1
  [rfi_detection] -> Inverter2/1
  Logical5/1 -> Register10/3, Register10/1
  Relational12/1 -> Logical6/2
  Inverter4/1 -> Logical6/1
  [rfi_detection] -> Inverter4/1
  Logical6/1 -> Register9/3, Register9/1
  ten_Gbe_v2/1(led_up) -> Terminator23/1
  Slice4/1 -> Subsystem2/3(din0), pipeline326/1(d)
  Slice9/1 -> Subsystem2/4(din1), pipeline323/1(d)
  Slice16/1 -> Subsystem2/5(din2), pipeline324/1(d)
  Slice17/1 -> pipeline325/1(d), Subsystem2/6(din3)
  power23/1 -> pipeline319/1(d)
  power20/1 -> pipeline320/1(d)
  power21/1 -> pipeline317/1(d)
  pipeline316/1(q) -> pipeline321/1(d)
  power22/1 -> pipeline318/1(d)
  pipeline320/1(q) -> adder_tree1/2(din1)
  pipeline317/1(q) -> adder_tree1/3(din2)
  pipeline321/1(q) -> adder_tree1/1(sync)
  pipeline318/1(q) -> adder_tree1/4(din3)
  pipeline319/1(q) -> adder_tree1/5(din4)
  pipeline327/1(q) -> pipeline316/1(d)
  pipeline326/1(q) -> power20/1
  pipeline325/1(q) -> power23/1
  pipeline323/1(q) -> power21/1
  pipeline324/1(q) -> power22/1
  ri_to_c7/1 -> power37/1
  ri_to_c6/1 -> power36/1
  simple_bram_vacc_0c_19/2(valid) -> pipeline455/1(d)
  simple_bram_vacc_0c_7/2(valid) -> pipeline456/1(d)
  ri_to_c5/1 -> power35/1
  ri_to_c4/1 -> power34/1
  simple_bram_vacc_0c_23/2(valid) -> pipeline454/1(d)
  pipeline524/1(q) -> pipeline414/1(d)
  simple_bram_vacc_0a_8/1(dout) -> pipeline335/1(d)
  simple_bram_vacc_0a_3/1(dout) -> pipeline334/1(d)
  simple_bram_vacc_0a_2/1(dout) -> pipeline333/1(d)
  pipeline490/1(q) -> pipeline336/1(d)
  simple_bram_vacc_0a_1/1(dout) -> pipeline332/1(d)
  simple_bram_vacc_0a_1/2(valid) -> pipeline337/1(d)
  simple_bram_vacc_0c_20/1(dout) -> pipeline330/1(d)
  simple_bram_vacc_0c_21/1(dout) -> pipeline331/1(d)
  simple_bram_vacc_0c_5/1(dout) -> pipeline329/1(d)
  simple_bram_vacc_0c_4/1(dout) -> pipeline328/1(d)
  simple_bram_vacc_0c_17/2(valid) -> pipeline458/1(d)
  pipeline329/1(q) -> Subsystem6/3(fft0_ch1)
  pipeline328/1(q) -> Subsystem6/2(fft0_ch0)
  pipeline331/1(q) -> Subsystem6/5(fft0_ch3)
  pipeline330/1(q) -> Subsystem6/4(fft0_ch2)
  pipeline335/1(q) -> Subsystem6/9(fft1_ch3)
  pipeline334/1(q) -> Subsystem6/8(fft1_ch2)
  pipeline333/1(q) -> Subsystem6/7(fft1_ch1)
  pipeline332/1(q) -> Subsystem6/6(fft1_ch0)
  pipeline336/1(q) -> Subsystem6/1(sync)
  pipeline337/1(q) -> Subsystem6/10(valid)
